simulink model "navigator"  (R2024b)
settings: Solver=FixedStepAuto  StartTime=0.0  StopTime=10.0  FixedStep=0.05  RelTol=1e-3
undefined symbols (not defined in the file or in its folder): CONSTANTS_RADIUS_OF_EARTH, GF_ACTION, GF_MAX_HOR_DIST, GF_MAX_VER_DIST
(part 2 of 2)

== stateflow chart navigator/Navigator ==
  state COMMAND [parallel]
    settings: executionOrder=1
    state CMD_DO_GO_AROUND [parallel]
      en:
      % 临时给输出赋值，后续删除
      o_pos_sp_triplet = i_pos_sp_triplet;
      o_mission_result.timestamp = uint64(getSimulationTime()*1e6);
      %
      settings: executionOrder=1
      state not_running
      state running
        en:
        publish_vehicle_command_ack(i_vehicle_command, VEHICLE_COMMAND.VEHICLE_CMD_RESULT_ACCEPTED);
      (default) -> COMMAND.CMD_DO_GO_AROUND.not_running
      COMMAND.CMD_DO_GO_AROUND.not_running -> COMMAND.CMD_DO_GO_AROUND.running : [i_vehicle_command.command == VEHICLE_COMMAND.VEHICLE_CMD_DO_GO_AROUND]
      COMMAND.CMD_DO_GO_AROUND.running -> COMMAND.CMD_DO_GO_AROUND.not_running : [i_vehicle_command.command ~= VEHICLE_COMMAND.VEHICLE_CMD_DO_GO_AROUND]
    state CMD_DO_REPOSITION [parallel]
      settings: executionOrder=2
      state not_running
      state running
        en:
        set_reposition_setpoint();
      (default) -> COMMAND.CMD_DO_REPOSITION.not_running
      COMMAND.CMD_DO_REPOSITION.not_running -> COMMAND.CMD_DO_REPOSITION.running : [i_vehicle_command.command == VEHICLE_COMMAND.VEHICLE_CMD_DO_REPOSITION ]
      COMMAND.CMD_DO_REPOSITION.running -> COMMAND.CMD_DO_REPOSITION.not_running : [i_vehicle_command.command ~= VEHICLE_COMMAND.VEHICLE_CMD_DO_REPOSITION]
    state CMD_NAV_TAKEOFF [parallel]
      settings: executionOrder=3
      state not_running
      state running
        en:
        % 前一航点
        if ((i_home_position.timestamp > 0) && i_home_position.valid_alt && i_home_position.valid_hpos && i_home_position.valid_lpos)
        g_takeoff_triplet.previous.valid = true;
        g_takeoff_triplet.previous.timestamp = uint64(getSimulationTime()*1e6);
        else
        g_takeoff_triplet.previous.valid = false;
        end
        g_takeoff_triplet.previous.lat = i_global_position.lat;
        g_takeoff_triplet.previous.lon = i_global_position.lon;
        g_takeoff_triplet.previous.alt = i_global_position.alt;
        g_takeoff_triplet.previous.yaw = i_local_position.heading;
        % 当前航点
        g_takeoff_triplet.current.valid = true;
        g_takeoff_triplet.current.timestamp = uint64(getSimulationTime()*1e6);
        g_takeoff_triplet.current.type = uint8(POSITION_SETPOINT.SETPOINT_TYPE_TAKEOFF);
        if isfinite(i_vehicle_command.param5) && isfinite(i_vehicle_command.param6)
        g_takeoff_triplet.current.lat = i_vehicle_command.param5;
        g_takeoff_triplet.current.lon = i_vehicle_command.param6;
        else
        g_takeoff_triplet.current.lat = i_global_position.lat;
        g_takeoff_triplet.current.lon = i_global_position.lon;
        end
        g_takeoff_triplet.current.alt = i_vehicle_command.param7;
        if ((i_home_position.timestamp > 0) && i_home_position.valid_alt && i_home_position.valid_hpos && i_home_position.valid_lpos)
        g_takeoff_triplet.current.yaw = i_vehicle_command.param4;
        else
        g_takeoff_triplet.current.yaw = i_local_position.heading;
        end
        g_takeoff_triplet.current.loiter_radius = NAV_LOITER_RAD;
        g_takeoff_triplet.current.loiter_direction = int8(1);
        % 下一航点
        g_takeoff_triplet.next.valid = false;
      (default) -> COMMAND.CMD_NAV_TAKEOFF.not_running
      COMMAND.CMD_NAV_TAKEOFF.not_running -> COMMAND.CMD_NAV_TAKEOFF.running : [i_vehicle_command.command == VEHICLE_COMMAND.VEHICLE_CMD_NAV_TAKEOFF]
      COMMAND.CMD_NAV_TAKEOFF.running -> COMMAND.CMD_NAV_TAKEOFF.not_running : [i_vehicle_command.command ~= VEHICLE_COMMAND.VEHICLE_CMD_NAV_TAKEOFF]
    state CMD_DO_CHANGE_SPEED [parallel]
      settings: executionOrder=4
      state not_running
      state running
        en:
        if (i_vehicle_command.param2 > eps)
        % 速度指令有效
        if (i_vehicle_status.vehicle_type == VEHICLE_STATUS.VEHICLE_TYPE_ROTARY_WING)
        g_mission_cruising_speed_mc = i_vehicle_command.param2;
        else
        g_mission_cruising_speed_fw = i_vehicle_command.param2;
        end
        else
        % 速度指令无效
        if (i_vehicle_status.vehicle_type == VEHICLE_STATUS.VEHICLE_TYPE_ROTARY_WING)
        g_mission_cruising_speed_mc = single(-1);
        else
        g_mission_cruising_speed_fw = single(-1);
        end
        % 设置油门指令
        if (i_vehicle_command.param3 > eps)
        g_mission_throttle = i_vehicle_command.param3 / 100;
        else
        g_mission_throttle = single(nan);
        end
        end
        publish_vehicle_command_ack(i_vehicle_command, VEHICLE_COMMAND.VEHICLE_CMD_RESULT_ACCEPTED);
      (default) -> COMMAND.CMD_DO_CHANGE_SPEED.not_running
      COMMAND.CMD_DO_CHANGE_SPEED.not_running -> COMMAND.CMD_DO_CHANGE_SPEED.running : [i_vehicle_command.command==VEHICLE_COMMAND.VEHICLE_CMD_DO_CHANGE_SPEED]
      COMMAND.CMD_DO_CHANGE_SPEED.running -> COMMAND.CMD_DO_CHANGE_SPEED.not_running : [i_vehicle_command.command~=VEHICLE_COMMAND.VEHICLE_CMD_DO_CHANGE_SPEED]
  state TRAFFIC [parallel]
    settings: executionOrder=2
  state GEOFENCE [parallel]
    settings: executionOrder=3
  state ACTION [parallel]
    en,du:
    switch uint8(i_vehicle_status.nav_state)
    case uint8(VEHICLE_STATUS.NAVIGATION_STATE_AUTO_MISSION)
    % g_pos_sp_triplet_published_invalid_once = false;
    % mission.set_execution_mode(mission_result_s::MISSION_EXECUTION_MODE_NORMAL);
    g_navigation_mode = VEHICLE_STATUS.NAVIGATION_STATE_AUTO_MISSION;
    case uint8(VEHICLE_STATUS.NAVIGATION_STATE_AUTO_LOITER)
    % g_pos_sp_triplet_published_invalid_once = false;
    g_navigation_mode = VEHICLE_STATUS.NAVIGATION_STATE_AUTO_LOITER;
    case uint8(VEHICLE_STATUS.NAVIGATION_STATE_AUTO_TAKEOFF)
    % g_pos_sp_triplet_published_invalid_once = false;
    g_navigation_mode = VEHICLE_STATUS.NAVIGATION_STATE_AUTO_TAKEOFF;
    case uint8(VEHICLE_STATUS.NAVIGATION_STATE_AUTO_LAND)
    % g_pos_sp_triplet_published_invalid_once = false;
    g_navigation_mode = VEHICLE_STATUS.NAVIGATION_STATE_AUTO_LAND;
    case uint8(VEHICLE_STATUS.NAVIGATION_STATE_AUTO_LANDENGFAIL)
    % g_pos_sp_triplet_published_invalid_once = false;
    g_navigation_mode = VEHICLE_STATUS.NAVIGATION_STATE_AUTO_LANDENGFAIL;
    case uint8(VEHICLE_STATUS.NAVIGATION_STATE_AUTO_LANDGPSFAIL)
    % g_pos_sp_triplet_published_invalid_once = false;
    g_navigation_mode = VEHICLE_STATUS.NAVIGATION_STATE_AUTO_LANDGPSFAIL;
    case uint8(VEHICLE_STATUS.NAVIGATION_STATE_AUTO_RTL)
    % g_pos_sp_triplet_published_invalid_once = false;
    % TODO
    otherwise
    g_navigation_mode = VEHICLE_STATUS.NAVIGATION_STATE_MAX;
    g_can_loiter_at_sp = false;
    end
    % 没有解锁不允许飞行
    if i_vehicle_status.arming_state ~= VEHICLE_STATUS.ARMING_STATE_ARMED
    g_navigation_mode = VEHICLE_STATUS.NAVIGATION_STATE_MAX;
    end
    % 记录当前导航状态
    %previous_nav_state = i_vehicle_status.nav_state;
    settings: executionOrder=4
    state LAND [parallel] [commented out]
      state on_disable [commented out]
      state on_active [commented out]
        state activation [commented out]
          en:
          set_land_item(true);
          o_mission_result.finished = false;
          g_mission_result_updated = true;
          % reset_mission_item_reached
          g_waypoint_position_reached = false;
          waypoint_yaw_reached_ = false;
          time_wp_reached_ = uint64(0);
          % convert mission item to current setpoint
          % 当前航点
          mission_item_ = NAV_STATE_ACTION.mission_apply_limitation(g_mission_item);
          NAV_STATE_ACTION.mission_item_to_position_setpoint(g_mission_item);
          % 前一航点
          o_pos_sp_triplet.previous.valid = false;
          % 下一航点
          o_pos_sp_triplet.next.valid = false;
          % 置标志位
          g_can_loiter_at_sp = false;
          g_pos_sp_triplet_updated = true;
        state active [commented out]
          en:
          % for VTOL update landing location during back transition
          o_pos_sp_triplet.current.lat = i_global_position.lat;
          o_pos_sp_triplet.current.lon = i_global_position.lon;
          g_pos_sp_triplet_updated = true;
        state Landed [commented out]
          en:
          o_mission_result.finished = true;
          g_mission_result_updated = true;
          NAV_STATE_ACTION.set_idle_item;
          NAV_STATE_ACTION.mission_item_to_position_setpoint(g_mission_item);
          g_pos_sp_triplet_updated = true;
        ACTION.LAND.on_active -> (junction 906) [commented out]
        (default) -> ACTION.LAND.on_active.activation [commented out]
        (junction 906) -> (junction 907) [commented out]
        (junction 906) -> ACTION.LAND.on_active.active [commented out] : % 飞机是vtol机型，并且处于过渡模式
            | [i_vehicle_status.is_vtol && i_vehicle_status.in_transition_mode]
        (junction 907) -> Landed [commented out] : % 飞机已经着陆
            | [land_detected.landed]
      (default) -> ACTION.LAND.on_disable [commented out]
      ACTION.LAND.on_disable -> ACTION.LAND.on_active [commented out] : [g_navigation_mode == NAVIGATION_MODE.land]
      ACTION.LAND.on_active -> ACTION.LAND.on_disable [commented out] : [g_navigation_mode ~= NAVIGATION_MODE.land]
    state LOITER [parallel] [commented out]
      state not_running [commented out]
        en,du:
        loiter_pos_set = false;
      state on_activation_active [commented out]
        state reposition [commented out]
          en:
          % rep的数据在navigator_main.cpp中处理
          o_pos_sp_triplet.current.velocity_valid = false;
          o_pos_sp_triplet.previous.yaw = i_local_position.heading;
          o_pos_sp_triplet.previous.lat = i_global_position.lat;
          o_pos_sp_triplet.previous.lon = i_global_position.lon;
          o_pos_sp_triplet.previous.alt = i_global_position.alt
          % 当前航路点用rep中表示
          o_pos_sp_triplet.current = g_reposition_triplet.current;
          % 下一个航路点无效
          o_pos_sp_triplet.next.valid = false;
          % 更新标志位
          g_can_loiter_at_sp = (o_pos_sp_triplet.current.type==POSITION_SETPOINT.SETPOINT_TYPE_LOITER);
          g_pos_sp_triplet_updated = true;
          % 设置reposition无效
          g_reposition_triplet.current.valid = false;
        state disarmed [commented out]
          en:
          loiter_pos_set = false;
        state set_loiter_pos [commented out]
          en:
          loiter_pos_set = true;
          % 若已着陆并上锁
          if ((i_vehicle_status.arming_state ~= VEHICLE_STATUS.ARMING_STATE_ARMED) && land_detected.landed)
          o_pos_sp_triplet.current.type = uint8(POSITION_SETPOINT.SETPOINT_TYPE_IDLE);
          g_can_loiter_at_sp = false;
          g_pos_sp_triplet_updated = true;
          loiter_pos_set = false;
          else
          g_mission_item.nav_cmd = uint16(NAVIGATION_CMD.NAV_CMD_LOITER_UNLIMITED);
          % set current mission item to loiter
          if (g_can_loiter_at_sp && o_pos_sp_triplet.current.valid)
          % 在当前的目标航点盘旋
          g_mission_item.lat = i_pos_sp_triplet.current.lat;
          g_mission_item.lon = i_pos_sp_triplet.current.lon;
          g_mission_item.altitude = i_pos_sp_triplet.current.alt;
          else
          % 在当前位置盘旋
          g_mission_item.lat = i_global_position.lat;
          g_mission_item.lon = i_global_position.lon;
          g_mission_item.altitude = i_global_position.alt;
          % （最小起飞高度 > 0 && item中的高度低于最小起飞的绝对高度），防止loiter高度在地面以下
          if (MIS_LTRMIN_ALT > 0) && (g_mission_item.altitude < i_home_position.alt + MIS_LTRMIN_ALT)
          g_mission_item.altitude = i_home_position.alt + MIS_LTRMIN_ALT;
          end
          end
          end
          g_mission_item.altitude_is_relative = false;
          g_mission_item.yaw = single(nan);
          g_mission_item.loiter_radius = NAV_LOITER_RAD;
          g_mission_item.acceptance_radius = navigator.get_acceptance_radius;
          g_mission_item.time_inside = single(0.0);
          g_mission_item.autocontinue = false;
          g_mission_item.origin = uint8(MISSION_ORIGIN.ONBOARD);
          % convert mission item to current setpoint
          o_pos_sp_triplet.previous.valid = false;
          % 当前航点
          o_pos_sp_triplet.current.velocity_valid = false;
          o_pos_sp_triplet.previous.velocity_valid = false;
          mission_item_ = NAV_STATE_ACTION.mission_apply_limitation(g_mission_item);
          NAV_STATE_ACTION.mission_item_to_position_setpoint(g_mission_item);
          %下一航点
          o_pos_sp_triplet.next.valid = false;
          % 更新标志位
          g_can_loiter_at_sp = (o_pos_sp_triplet.current.type==POSITION_SETPOINT.SETPOINT_TYPE_LOITER);
          g_pos_sp_triplet_updated = true;
        (default) -> (junction 846) [commented out]
        reposition -> reposition [commented out] : [g_reposition_triplet.current.valid]
        reposition -> disarmed [commented out] : [i_vehicle_status.arming_state ~= VEHICLE_STATUS.ARMING_STATE_ARMED]
        (junction 846) -> reposition [commented out] : [g_reposition_triplet.current.valid]
        (junction 846) -> (junction 847) [commented out]
        set_loiter_pos -> reposition [commented out] : [g_reposition_triplet.current.valid]
        (junction 847) -> set_loiter_pos [commented out]
      (default) -> ACTION.LOITER.not_running [commented out]
      ACTION.LOITER.not_running -> ACTION.LOITER.on_activation_active [commented out] : [g_navigation_mode == NAVIGATION_MODE.loiter]
      ACTION.LOITER.on_activation_active -> ACTION.LOITER.not_running [commented out] : [g_navigation_mode ~= NAVIGATION_MODE.loiter]
    state RTL [parallel] [commented out]
      state not_running [commented out]
        en,du:
        rtl_state = RTL_STATE.NONE;
        find_RTL_destination;
      state running [commented out]
        en:
        % TO DO: output RTL message, home / mission / safe point
        % 垂起旋翼阶段取消mission方式的降落，因为此处已经不是mission模式了
        deny_mission_landing_ = i_vehicle_status.is_vtol && (i_vehicle_status.vehicle_type == VEHICLE_STATUS.VEHICLE_TYPE_ROTARY_WING);
        get_rtl_alt_and_rad;
        print_des_type;
        state RTL_STATE_CLIMB [commented out]
          en:
          rtl_state = RTL_STATE.CLIMB;
          climb_and_return_done_ = false;
          g_can_loiter_at_sp = false;
          % 在当前位置爬升至指定高度
          if (i_vehicle_status.vehicle_type == VEHICLE_STATUS.VEHICLE_TYPE_ROTARY_WING)
          % 如果多旋翼则直接爬升到给定高度
          g_mission_item.nav_cmd = uint16(NAVIGATION_CMD.NAV_CMD_WAYPOINT);
          else
          %如果是固定翼，则盘旋上升到给定高度
          g_mission_item.nav_cmd = uint16(NAVIGATION_CMD.NAV_CMD_LOITER_TO_ALT);
          end
          g_mission_item.lat = i_global_position.lat;
          g_mission_item.lon = i_global_position.lon;
          g_mission_item.altitude = rtl_alt;
          g_mission_item.altitude_is_relative = false;
          g_mission_item.yaw = i_local_position.heading;
          g_mission_item.acceptance_radius = navigator.get_acceptance_radius;
          g_mission_item.time_inside = single(0);
          g_mission_item.autocontinue = true;
          g_mission_item.origin =uint8(MISSION_ORIGIN.ONBOARD);
          sprintf("RTL: climb to %f m (%f m above destination) \t", double(rtl_alt), double(rtl_alt - destination.alt))
          % mavlink_log_info(_navigator->get_mavlink_log_pub(), "RTL: climb to %d m (%d m above destination)\t",(int)ceilf(_rtl_alt), (int)ceilf(_rtl_alt - _destination.alt));
          % Reset all reached flags
          g_waypoint_position_reached = false;
          waypoint_yaw_reached_ = false;
          time_wp_reached_ = uint64(0);
          % TO DO: issue_command
          % 更新当前航点
          mission_item_ = NAV_STATE_ACTION.mission_apply_limitation(g_mission_item);
          NAV_STATE_ACTION.mission_item_to_position_setpoint(g_mission_item);
          g_pos_sp_triplet_updated = true;
        state RTL_STATE_RETURN [commented out]
          en:
          rtl_state = RTL_STATE.RETURN;
          climb_and_return_done_ = false;
          g_can_loiter_at_sp = false;
          % 返航至目标航点
          g_mission_item.nav_cmd = uint16(NAVIGATION_CMD.NAV_CMD_WAYPOINT);
          g_mission_item.lat = destination.lat;
          g_mission_item.lon = destination.lon;
          g_mission_item.altitude = rtl_alt;
          g_mission_item.altitude_is_relative = false;
          destination_dist = navigator.get_distance_2_next_waypoint(destination.lat, destination.lon, i_global_position.lat, i_global_position.lon);
          if (destination_dist < RTL_MIN_DIST)
          % 如果离着陆点很近，则采用着陆的航向
          g_mission_item.yaw = destination.yaw;
          else
          % 否则机头指向着陆点
          g_mission_item.yaw = navigator.get_bearing_2_next_waypoint(i_global_position.lat, i_global_position.lon, destination.lat, destination.lon);
          end
          g_mission_item.acceptance_radius = navigator.get_acceptance_radius;
          g_mission_item.time_inside = single(0);
          g_mission_item.autocontinue = true;
          g_mission_item.origin = uint8(MISSION_ORIGIN.ONBOARD);
          sprintf("RTL: return at %f m (%f m above destination) \t", double(g_mission_item.altitude), double(g_mission_item.altitude - destination.alt))
          % Reset all reached flags
          g_waypoint_position_reached = false;
          waypoint_yaw_reached_ = false;
          time_wp_reached_ = uint64(0);
          % TO DO: issue_command
          % 更新当前航点
          mission_item_ = NAV_STATE_ACTION.mission_apply_limitation(g_mission_item);
          NAV_STATE_ACTION.mission_item_to_position_setpoint(g_mission_item);
          g_pos_sp_triplet_updated = true;
        state RTL_STATE_DESCEND [commented out]
          en:
          rtl_state = RTL_STATE.DESCEND;
          climb_and_return_done_ = true;
          g_can_loiter_at_sp = false;
          % 下降至指定高度
          g_mission_item.nav_cmd = uint16(NAVIGATION_CMD.NAV_CMD_LOITER_TO_ALT);
          g_mission_item.lat = destination.lat;
          g_mission_item.lon = destination.lon;
          g_mission_item.altitude = min([destination.alt + RTL_DESCEND_ALT, i_global_position.alt, rtl_alt]);
          g_mission_item.altitude_is_relative = false;
          % Except for vtol which might be still off here and should point towards this location.
          d_current = navigator.get_distance_2_next_waypoint(i_global_position.lat, i_global_position.lon, g_mission_item.lat, g_mission_item.lon);
          if (i_vehicle_status.is_vtol && (d_current > navigator.get_acceptance_radius))
          g_mission_item.yaw = navigator.get_bearing_2_next_waypoint(i_global_position.lat, i_global_position.lon, g_mission_item.lat, g_mission_item.lon);
          else
          g_mission_item.yaw = destination.yaw;
          end
          if (i_vehicle_status.is_vtol)
          g_mission_item.loiter_radius = rtl_loiter_rad;
          end
          g_mission_item.acceptance_radius = navigator.get_acceptance_radius;
          g_mission_item.time_inside = single(0);
          g_mission_item.autocontinue = true;
          g_mission_item.origin = uint8(MISSION_ORIGIN.ONBOARD);
          % Disable previous setpoint to prevent drift.
          o_pos_sp_triplet.previous.valid = false;
          sprintf("RTL: descend to %f m (%f m above destination) \t", double(g_mission_item.altitude), double(g_mission_item.altitude - destination.alt))
          % Reset all reached flags
          g_waypoint_position_reached = false;
          waypoint_yaw_reached_ = false;
          time_wp_reached_ = uint64(0);
          % TO DO: issue_command
          % 更新当前航点
          mission_item_ = NAV_STATE_ACTION.mission_apply_limitation(g_mission_item);
          NAV_STATE_ACTION.mission_item_to_position_setpoint(g_mission_item);
          g_pos_sp_triplet_updated = true;
        state RTL_STATE_LOITER [commented out]
          en:
          rtl_state = RTL_STATE.LOITER;
          climb_and_return_done_ = true;
          g_can_loiter_at_sp = true;
          % Don't change altitude.
          g_mission_item.lat = destination.lat;
          g_mission_item.lon = destination.lon;
          g_mission_item.altitude = min([destination.alt + RTL_DESCEND_ALT, i_global_position.alt, rtl_alt]);
          g_mission_item.altitude_is_relative = false;
          g_mission_item.yaw = destination.yaw;
          g_mission_item.loiter_radius = NAV_LOITER_RAD;
          g_mission_item.acceptance_radius = navigator.get_acceptance_radius;
          g_mission_item.time_inside = max(RTL_LAND_DELAY, single(0.0));
          g_mission_item.autocontinue = (RTL_LAND_DELAY > eps);
          g_mission_item.origin = uint8(MISSION_ORIGIN.ONBOARD);
          if (RTL_LAND_DELAY > eps)
          g_mission_item.nav_cmd = uint16(NAVIGATION_CMD.NAV_CMD_LOITER_TIME_LIMIT)
          sprintf("RTL: loiter %f. \t", double(g_mission_item.time_inside));
          %mavlink_log_info(_navigator->get_mavlink_log_pub(), "RTL: loiter %.1fs\t", (double)get_time_inside(_mission_item));
          %events::send<float>(events::ID("rtl_loiter"), events::Log::Info, "RTL: loiter {1:.1}s", get_time_inside(_mission_item));
          else
          g_mission_item.nav_cmd = uint16(NAVIGATION_CMD.NAV_CMD_LOITER_UNLIMITED);
          sprintf("RTL: completed, loitering. \t")
          %mavlink_log_info(_navigator->get_mavlink_log_pub(), "RTL: completed, loitering\t");
          %events::send(events::ID("rtl_completed_loiter"), events::Log::Info, "RTL: completed, loitering");
          end
          % Reset all reached flags
          g_waypoint_position_reached = false;
          waypoint_yaw_reached_ = false;
          time_wp_reached_ = uint64(0);
          % TO DO: issue_command
          % 更新当前航点
          mission_item_ = NAV_STATE_ACTION.mission_apply_limitation(g_mission_item);
          NAV_STATE_ACTION.mission_item_to_position_setpoint(g_mission_item);
          g_pos_sp_triplet_updated = true;
        state RTL_STATE_LAND [commented out]
          en:
          rtl_state = RTL_STATE.LANDING;
          climb_and_return_done_ = true;
          g_can_loiter_at_sp = false;
          % Land at destination.
          g_mission_item.nav_cmd = uint16(NAVIGATION_CMD.NAV_CMD_LAND);
          g_mission_item.lat = destination.lat;
          g_mission_item.lon = destination.lon;
          g_mission_item.yaw = destination.yaw;
          g_mission_item.altitude = destination.alt;
          g_mission_item.altitude_is_relative = false;
          g_mission_item.acceptance_radius = navigator.get_acceptance_radius;
          g_mission_item.time_inside = single(0);
          g_mission_item.autocontinue = true;
          g_mission_item.origin = uint8(MISSION_ORIGIN.ONBOARD);
          %g_mission_item.land_precision = RTL_PLD_MD;
          %if (g_mission_item.land_precision == 1)
          %_navigator->get_precland()->set_mode(PrecLandMode::Opportunistic);
          %_navigator->get_precland()->on_activation();
          %elseif (g_mission_item.land_precision == 2)
          %_navigator->get_precland()->set_mode(PrecLandMode::Required);
          %_navigator->get_precland()->on_activation();
          %end
          sprintf("RTL: land at destination")
          %mavlink_log_info(_navigator->get_mavlink_log_pub(), "RTL: land at destination\t");
          % %events::send(events::ID("rtl_land_at_destination"), events::Log::Info, "RTL: land at destination");
          % Reset all reached flags
          g_waypoint_position_reached = false;
          waypoint_yaw_reached_ = false;
          time_wp_reached_ = uint64(0);
          % TO DO: issue_command
          % 更新当前航点
          mission_item_ = NAV_STATE_ACTION.mission_apply_limitation(g_mission_item);
          NAV_STATE_ACTION.mission_item_to_position_setpoint(g_mission_item);
          g_pos_sp_triplet_updated = true;
        state RTL_MOVE_TO_LAND_HOVER_VTOL [commented out]
          en:
          rtl_state = RTL_STATE.MOVE_TO_LAND_HOVER_VTOL;
          climb_and_return_done_ = true;
          g_can_loiter_at_sp = false;
          %
          g_mission_item.nav_cmd = uint16(NAVIGATION_CMD.NAV_CMD_WAYPOINT);
          g_mission_item.lat = destination.lat;
          g_mission_item.lon = destination.lon;
          g_mission_item.altitude = min([destination.alt + RTL_DESCEND_ALT, i_global_position.alt, rtl_alt]);
          g_mission_item.altitude_is_relative = false;
          g_mission_item.yaw = navigator.get_bearing_2_next_waypoint(i_global_position.lat, i_global_position.lon, g_mission_item.lat, g_mission_item.lon);
          g_mission_item.acceptance_radius = navigator.get_acceptance_radius;
          g_mission_item.origin = uint8(MISSION_ORIGIN.ONBOARD);
          % Reset all reached flags
          g_waypoint_position_reached = false;
          waypoint_yaw_reached_ = false;
          time_wp_reached_ = uint64(0);
          % TO DO: issue_command
          % 更新当前航点
          mission_item_ = NAV_STATE_ACTION.mission_apply_limitation(g_mission_item);
          NAV_STATE_ACTION.mission_item_to_position_setpoint(g_mission_item);
          g_pos_sp_triplet_updated = true;
        state RTL_STATE_TRANSITION_TO_MC [commented out]
          en:
          rtl_state = RTL_STATE.TRANSITION_TO_MC;
          climb_and_return_done_ = true;
          g_can_loiter_at_sp = false;
          % 设置固定翼切换到旋翼的过渡点
          g_mission_item.nav_cmd = uint16(NAVIGATION_CMD.NAV_CMD_DO_VTOL_TRANSITION);
          % params 是union联合体
          g_mission_item.time_inside = single(VTOL_VEHICLE_STATUS.VEHICLE_VTOL_STATE_MC);
          g_mission_item.acceptance_radius = single(0.0);
          g_mission_item.yaw = i_local_position.heading;
          g_mission_item.autocontinue = true;
          % Reset all reached flags
          g_waypoint_position_reached = false;
          waypoint_yaw_reached_ = false;
          time_wp_reached_ = uint64(0);
          % TO DO: issue_command
          % 更新当前航点
          mission_item_ = NAV_STATE_ACTION.mission_apply_limitation(g_mission_item);
          NAV_STATE_ACTION.mission_item_to_position_setpoint(g_mission_item);
          g_pos_sp_triplet_updated = true;
        state RTL_STATE_HEAD_TO_CENTER [commented out]
          en:
          rtl_state = RTL_STATE.HEAD_TO_CENTER;
          climb_and_return_done_ = true;
          g_can_loiter_at_sp = false;
          %
          g_mission_item.nav_cmd = uint16(NAVIGATION_CMD.NAV_CMD_WAYPOINT);
          g_mission_item.lat = destination.lat;
          g_mission_item.lon = destination.lon;
          g_mission_item.altitude = min([destination.alt + RTL_DESCEND_ALT, i_global_position.alt, rtl_alt]);
          g_mission_item.altitude_is_relative = false;
          g_mission_item.yaw = navigator.get_bearing_2_next_waypoint(i_global_position.lat, i_global_position.lon, g_mission_item.lat, g_mission_item.lon);
          g_mission_item.acceptance_radius = navigator.get_acceptance_radius;
          g_mission_item.time_inside = single(0);
          g_mission_item.autocontinue = true;
          g_mission_item.origin = uint8(MISSION_ORIGIN.ONBOARD);
          % Disable previous setpoint to prevent drift.
          o_pos_sp_triplet.previous.valid = false;
          % Reset all reached flags
          g_waypoint_position_reached = false;
          waypoint_yaw_reached_ = false;
          time_wp_reached_ = uint64(0);
          % TO DO: issue_command
          % 更新当前航点
          mission_item_ = NAV_STATE_ACTION.mission_apply_limitation(g_mission_item);
          NAV_STATE_ACTION.mission_item_to_position_setpoint(g_mission_item);
          g_pos_sp_triplet_updated = true;
        state RTL_STATE_LANDED [commented out]
          en:
          rtl_state = RTL_STATE.LANDED
          climb_and_return_done_ = true;
          g_can_loiter_at_sp = false;
          %
          NAV_STATE_ACTION.set_idle_item;
          rtl_alt_min_ = false;
          % Reset all reached flags
          g_waypoint_position_reached = false;
          waypoint_yaw_reached_ = false;
          time_wp_reached_ = uint64(0);
          % TO DO: issue_command
          % 更新当前航点
          mission_item_ = NAV_STATE_ACTION.mission_apply_limitation(g_mission_item);
          NAV_STATE_ACTION.mission_item_to_position_setpoint(g_mission_item);
          g_pos_sp_triplet_updated = true;
        (default) -> RTL_STATE_DESCEND [commented out] : % 如果rtl降落点类型为MISSION_LANDING，并且飞行器处于正在降落的过程中
            | [destination.type == RTL_DESTINATION_TYPE.MISSION_LANDING && ...
            | mission_landing_in_progress_]
        (default) -> RTL_STATE_CLIMB [commented out] : % 如果飞行器的高度低于预设的降落高度
            | [i_global_position.alt < ((destination.alt + RTL_RETURN_ALT) || ...
            | rtl_alt_min_)]
        (default) -> RTL_STATE_RETURN [commented out]
        RTL_STATE_CLIMB -> RTL_STATE_RETURN [commented out] : [NAV_STATE_ACTION.is_mission_item_reached(g_mission_item)]
        RTL_STATE_RETURN -> (junction 800) [commented out] : [NAV_STATE_ACTION.is_mission_item_reached(g_mission_item)]
        (junction 800) -> RTL_STATE_DESCEND [commented out] : [(RTL_LAND_DELAY < -0.01 || RTL_LAND_DELAY > 0.01) || ...
            | (i_vehicle_status.is_vtol && i_vehicle_status.vehicle_type == VEHICLE_STATUS.VEHICLE_TYPE_FIXED_WING)]
        (junction 800) -> (junction 801) [commented out]
        RTL_STATE_DESCEND -> (junction 802) [commented out] : [NAV_STATE_ACTION.is_mission_item_reached(g_mission_item)]
        (junction 802) -> (junction 801) [commented out]
        (junction 802) -> (junction 803) [commented out] : [i_vehicle_status.is_vtol && ...
            | i_vehicle_status.vehicle_type == VEHICLE_STATUS.VEHICLE_TYPE_FIXED_WING]
        (junction 801) -> (junction 805) [commented out]
        (junction 802) -> RTL_STATE_LOITER [commented out] : [RTL_LAND_DELAY < -0.01 || RTL_LAND_DELAY > 0.01]
        (junction 803) -> RTL_STATE_HEAD_TO_CENTER [commented out]
        RTL_STATE_LOITER -> (junction 805) [commented out] : [NAV_STATE_ACTION.is_mission_item_reached(g_mission_item)]
        (junction 805) -> (junction 804) [commented out]
        (junction 804) -> RTL_STATE_LAND [commented out]
        RTL_STATE_TRANSITION_TO_MC -> RTL_MOVE_TO_LAND_HOVER_VTOL [commented out] : [NAV_STATE_ACTION.is_mission_item_reached(g_mission_item)]
        RTL_MOVE_TO_LAND_HOVER_VTOL -> RTL_STATE_LAND [commented out] : [NAV_STATE_ACTION.is_mission_item_reached(g_mission_item)]
        RTL_STATE_HEAD_TO_CENTER -> RTL_STATE_TRANSITION_TO_MC [commented out] : [NAV_STATE_ACTION.is_mission_item_reached(g_mission_item)]
        RTL_STATE_LAND -> RTL_STATE_LANDED [commented out] : [NAV_STATE_ACTION.is_mission_item_reached(g_mission_item)]
        (default) -> RTL_STATE_LANDED [commented out] : % 飞行器已经着陆
            | [land_detected.landed]
      (default) -> ACTION.RTL.not_running [commented out]
      ACTION.RTL.not_running -> ACTION.RTL.running [commented out] : [g_navigation_mode == NAVIGATION_MODE.rtl]
      ACTION.RTL.running -> ACTION.RTL.not_running [commented out] : [g_navigation_mode ~= NAVIGATION_MODE.rtl]
    state TAKEOFF [parallel]
      settings: executionOrder=1
      state on_disable
      state on_active
        state takeoff_entry
          en:
          set_takeoff_position()
        state takeoff_finished
          en:
          set_takeoff_finished()
        (default) -> takeoff_entry
        takeoff_finished -> takeoff_entry : [g_takeoff_triplet.current.valid]
        takeoff_entry -> takeoff_finished : [is_mission_item_reached()]
      (default) -> ACTION.TAKEOFF.on_disable
      ACTION.TAKEOFF.on_disable -> ACTION.TAKEOFF.on_active : [g_navigation_mode==VEHICLE_STATUS.NAVIGATION_STATE_AUTO_TAKEOFF]
      ACTION.TAKEOFF.on_active -> ACTION.TAKEOFF.on_disable : [g_navigation_mode~=VEHICLE_STATUS.NAVIGATION_STATE_AUTO_TAKEOFF]
    state ENGINE_FAILURE [parallel] [commented out]
      state not_running [commented out]
        en,du:
        % ef_state: engine failure state
        ef_state = EFSTATE.EF_STATE_NONE;
      state on_activation_active [commented out]
        state activation [commented out]
          en:
          ef_state = EFSTATE.EF_STATE_NONE;
          advance_ef;
          set_ef_item;
        state active [commented out]
          en:
          advance_ef;
          set_ef_item;
        ACTION.ENGINE_FAILURE.on_activation_active -> ACTION.ENGINE_FAILURE.on_activation_active.active [commented out] : [NAV_STATE_ACTION.is_mission_item_reached(g_mission_item)]
        (default) -> ACTION.ENGINE_FAILURE.on_activation_active.activation [commented out]
      (default) -> ACTION.ENGINE_FAILURE.not_running [commented out]
      ACTION.ENGINE_FAILURE.not_running -> ACTION.ENGINE_FAILURE.on_activation_active [commented out] : [g_navigation_mode == NAVIGATION_MODE.engineFailure]
      ACTION.ENGINE_FAILURE.on_activation_active -> ACTION.ENGINE_FAILURE.not_running [commented out] : [g_navigation_mode ~= NAVIGATION_MODE.engineFailure]
    state MISSION [parallel] [commented out]
      state not_running [commented out]
      state running [commented out]
        en:
      (default) -> ACTION.MISSION.not_running [commented out]
      ACTION.MISSION.not_running -> ACTION.MISSION.running [commented out] : [g_navigation_mode == NAVIGATION_MODE.mission]
      ACTION.MISSION.running -> ACTION.MISSION.not_running [commented out] : [g_navigation_mode ~= NAVIGATION_MODE.mission]
    state GPS_FAILURE [parallel] [commented out]
      state not_running [commented out]
        en,du:
        % 仅在setpoint移动时重置GPS_FAILURE状态
        if (~g_can_loiter_at_sp)
        gpsf_state = GPSFSTATE.GPSF_STATE_NONE;
        end
      state on_activation_active [commented out]
        state activation [commented out]
          en:
          gpsf_state = GPSFSTATE.GPSF_STATE_NONE;
          timestamp_activation = uint64(getSimulationTime()*1e6);
          advance_gpsf;
          set_gpsf_item;
        state active [commented out]
          en:
          switch (gpsf_state)
          case GPSFSTATE.GPSF_STATE_LOITER
          % 在这种情况下，不会运行位置控制器；所以navigator在这里发布姿态的setpoint
          % att_sp.timestamp = uint64(getSimulationTime()*1e6);
          % att_sp.roll_body = single(deg2rad(NAV_GPSF_R));
          % att_sp.pitch_body = single(deg2rad(NAV_GPSF_P));
          % att_sp.thrust_body(1) = NAV_GPSF_TR;
          % att_sp.q_d = euler_to_quat(att_sp.roll_body, att_sp.pitch_body, 0);
          % TO DO: publish att_sp
          %
          % measure time
          if (NAV_GPSF_LT > eps) && ((uint64(getSimulationTime()*1e6) - timestamp_activation) > NAV_GPSF_LT)
          sprintf("GPS not recovered, switching to next failure state. \n")
          advance_gpsf;
          end
          case GPSFSTATE.GPSF_STATE_TERMINATE
          set_gpsf_item;
          advance_gpsf;
          otherwise
          end
        ACTION.GPS_FAILURE.on_activation_active -> ACTION.GPS_FAILURE.on_activation_active.active [commented out]
        (default) -> ACTION.GPS_FAILURE.on_activation_active.activation [commented out]
      (default) -> ACTION.GPS_FAILURE.not_running [commented out]
      ACTION.GPS_FAILURE.not_running -> ACTION.GPS_FAILURE.on_activation_active [commented out] : [g_navigation_mode == NAVIGATION_MODE.gpsFailure]
      ACTION.GPS_FAILURE.on_activation_active -> ACTION.GPS_FAILURE.not_running [commented out] : [g_navigation_mode ~= NAVIGATION_MODE.gpsFailure]
  data: phi function_input; theta function_input; psi function_input; q0 function_output; q1 function_output; q2 function_output; q3 function_output; lat function_input; lon function_input; alt function_input; inside function_output; at_current_location function_input; loiter_pos_set local boolean size=1 =false; destination_check_time local uint64 size=1 =uint64(0); destination_dist local single; d_current local single size=1; rtl_state local Enum: PX4_RTL_STATE size=1; rtl_loiter_rad local single size=1; rtl_alt local single size=1; destination local Bus: px4_rtl_position size=1; deny_mission_landing_ local boolean size=1 =false; mission_landing_in_progress_ local boolean size=1 =false; climb_and_return_done_ local boolean size=1 =false; ef_state local Enum: PX4_EFSTATE size=1; destination_check_time local uint64 size=1 =uint64(0); rtl_state local Enum: PX4_RTL_STATE size=1; rtl_loiter_rad local single size=1; rtl_alt local single size=1; destination local Bus: px4_rtl_position; gpsf_state local Enum: PX4_GPSFSTATE size=1; timestamp_activation local uint64 size=1; time function_output; item function_input; abs_altitude function_input; alt function_output; isreached function_output; min_clearance function_input; item function_output; at_current_location function_input; g_waypoint_position_reached local boolean size=1 =false; waypoint_yaw_reached_ local boolean size=1 =false; time_wp_reached_ local uint64 size=1 =uint64(0); lat_now function_input; lon_now function_input; lat_next function_input; lon_next function_input; dist function_output; lat_now function_input; lon_now function_input; lat_next function_input; lon_next function_input; bearing function_output; speed function_output; radius function_output; radius function_output single; speed function_input; radius function_output single; radius function_output; radius function_output; mission_item_yaw function_input; yaw function_output; cmd function_input; result function_input; throttle function_output single; i_vehicle_command input Bus: vehicle_command_s size=1; i_global_position input Bus: vehicle_global_position_s size=1; i_local_position input Bus: vehicle_local_position_s size=1; i_vehicle_status input Bus: vehicle_status_s size=1; RTL_RETURN_ALT parameter size=1; RTL_CONE_ANG parameter size=1; RTL_LOITER_RAD parameter size=1; NAV_ACC_RAD parameter size=1; g_pos_sp_triplet_updated local boolean size=1; i_land_detected input Bus: vehicle_land_detected_s size=1; i_pos_sp_triplet input Bus: position_setpoint_triplet_s size=1; i_home_position input Bus: home_position_s size=1; NAV_LOITER_RAD parameter size=1; i_pos_ctrl_status input Bus: position_controller_status_s size=1; o_pos_sp_triplet output Bus: position_setpoint_triplet_s size=1; MIS_LTRMIN_ALT parameter size=1; g_mission_throttle local single size=1 =single(nan); g_mission_cruising_speed_mc local single size=1 =single(-1.0); g_mission_cruising_speed_fw local single size=1 =single(-1.0); g_reposition_triplet local Bus: position_setpoint_triplet_s size=1; g_takeoff_triplet local Bus: position_setpoint_triplet_s size=1; MIS_TAKEOFF_ALT parameter size=1; o_mission_result output Bus: mission_result_s size=1; NAV_GPSF_R parameter size=1; NAV_GPSF_P parameter size=1; NAV_GPSF_TR parameter size=1; NAV_GPSF_LT parameter size=1; CONSTANTS_RADIUS_OF_EARTH parameter single size=1; RTL_MIN_DIST parameter single size=1; g_rtl_alt_min local boolean size=1 =false; RTL_DESCEND_ALT parameter size=1; RTL_LAND_DELAY parameter size=1; RTL_PLD_MD parameter size=1; RTL_TYPE parameter size=1; VT_B_DEC_MSS parameter size=1; VT_B_REV_DEL parameter size=1; MIS_YAW_ERR parameter size=1; MIS_YAW_TMT parameter size=1; NAV_FW_ALTL_RAD parameter size=1; NAV_FW_ALT_RAD parameter size=1; NAV_MC_ALT_RAD parameter size=1; GF_ACTION parameter size=1; MPC_JERK_AUTO parameter size=1; MPC_ACC_HOR parameter size=1; g_navigation_mode local Enum: VEHICLE_STATUS size=1; g_mission_item local Bus: mission_route_point_s size=1; g_mission_result_updated local boolean size=1 =false; g_can_loiter_at_sp local boolean size=1 =false; o_command_ack output Bus: vehicle_command_ack_s; MISSION_ORIGIN_ONBOARD constant uint8 size=1 =1; MISSION_ORIGIN_MAVLINK constant uint8 size=1 =0
  function [q0,q1,q2,q3] = eul_to_quat(phi,theta,psi):
    | function [q0,q1,q2,q3] = eul_to_quat(phi,theta,psi)
    | [q0,q1,q2,q3] = euler2quat(phi,theta,psi);
    | end
  function set_reposition_setpoint:
    | function set_reposition_setpoint
    | 
    | %% 判断reposition是否在禁飞区内
    | reposition_valid = true;
    | if (GF_ACTION ~= GEOFENCE_RESULT.GF_ACTION_NONE &&  GF_ACTION ~= GEOFENCE_RESULT.GF_ACTION_WARN)
    |     if isfinite(i_vehicle_command.param5) && isfinite(i_vehicle_command.param6)
    |         lat = i_vehicle_command.param5;
    |         lon = i_vehicle_command.param6;
    | 
    |         if isfinite(i_vehicle_command.param7)
    |             alt = i_vehicle_command.param7;
    |         else
    |             alt = i_global_position.alt;
    |         end
    | 
    |         reposition_valid = GEOFENCE.checkAll(lat, lon, alt);
    |     end
    | end
    | 
    | if ~reposition_valid
    |     %mavlink_log_critical(&_mavlink_log_pub, "Reposition is outside geofence\t");
    |     %events::send(events::ID("navigator_reposition_outside_geofence"), {events::Log::Error, events::LogInternal::Info},
    |     %"Reposition is outside geofence");
    | end
    | 
    | %% 初始化上个航点
    | g_reposition_triplet.previous.valid = true;
    | g_reposition_triplet.previous.timestamp = uint64(getSimulationTime()*1e6);
    | g_reposition_triplet.previous.lat = i_global_position.lat;
    | g_reposition_triplet.previous.lon = i_global_position.lon;
    | g_reposition_triplet.previous.alt = i_global_position.alt;
    | g_reposition_triplet.previous.yaw = i_local_position.heading;
    | 
    | %% 初始化当前航点
    | g_reposition_triplet.current.valid = true;
    | g_reposition_triplet.current.timestamp = uint64(getSimulationTime()*1e6);
    | g_reposition_triplet.current.loiter_radius = NAV_LOITER_RAD;
    | g_reposition_triplet.current.loiter_direction = int8(1);
    | g_reposition_triplet.current.type = uint8(POSITION_SETPOINT.SETPOINT_TYPE_LOITER);
    | 
    | % 如果没有速度参数，使用默认值
    | if (i_vehicle_command.param1 <= 0 || ~isfinite(i_vehicle_command.param1))
    |     g_reposition_triplet.current.cruising_speed = get_cruising_speed();
    | else
    |     g_reposition_triplet.current.cruising_speed = i_vehicle_command.param1;
    | end
    | % 油门
    | g_reposition_triplet.current.cruising_throttle = get_cruising_throttle();
    | % 提前量
    | g_reposition_triplet.current.acceptance_radius = get_acceptance_radius();
    | % 偏航角
    | if isfinite(i_vehicle_command.param4)
    |     g_reposition_triplet.current.yaw = i_vehicle_command.param4;
    |     g_reposition_triplet.current.yaw_valid = true;
    | else
    |     g_reposition_triplet.current.yaw = single(nan);
    |     g_reposition_triplet.current.yaw_valid = false;
    | end
    | % 经纬高
    | if isfinite(i_vehicle_command.param5) && isfinite(i_vehicle_command.param6)
    |     % 经纬度有效
    |     g_reposition_triplet.current.lat = i_vehicle_command.param5;
    |     g_reposition_triplet.current.lon = i_vehicle_command.param6;
    |     if isfinite(i_vehicle_command.param7)
    |         g_reposition_triplet.current.alt = i_vehicle_command.param7;
    |     else
    |         g_reposition_triplet.current.alt = i_global_position.alt;
    |     end
    | elseif i_vehicle_command.param7
    |     % 经纬度无效，高度有效
    |     g_reposition_triplet.current.lat = i_pos_sp_triplet.current.lat;
    |     g_reposition_triplet.current.lon = i_pos_sp_triplet.current.lon;
    |     g_reposition_triplet.current.alt = i_vehicle_command.param7;
    | else
    |     % 经纬高均无效
    |     g_reposition_triplet.current.alt = i_global_position.alt;
    | 
    |     if i_vehicle_status.vehicle_type == VEHICLE_STATUS.VEHICLE_TYPE_ROTARY_WING && i_pos_sp_triplet.current.type ~= uint8(POSITION_SETPOINT.SETPOINT_TYPE_TAKEOFF)
    |         % 多旋翼计算刹车距离，确定悬停位置
    |         course_over_ground = atan2(i_local_position.vy, i_local_position.vx);
    |         velocity_hor_abs = sqrt(i_local_position.vx^2 + i_local_position.vy^2);
    |         multirotor_braking_distance = velocity_hor_abs * (velocity_hor_abs / (2 * MPC_ACC_HOR) + (0.6 * MPC_JERK_AUTO) / MPC_JERK_AUTO);
    | 
    |         [g_reposition_triplet.current.lat, g_reposition_triplet.current.lon] = waypoint_from_heading_and_distance(i_global_position.lat, i_global_position.lon,...
    |             course_over_ground, multirotor_braking_distance);
    |         g_reposition_triplet.current.yaw = i_local_position.heading;
    |         g_reposition_triplet.current.yaw_valid = true;
    |     else
    |         % 固定翼使用当前位置进行盘旋
    |         g_reposition_triplet.current.lat = i_global_position.lat;
    |         g_reposition_triplet.current.lon = i_global_position.lon;
    |     end
    | end
    | 
    | %% 初始化下个航点
    | g_reposition_triplet.next.valid = false;
    | 
    | end
  function inside = checkAll(lat, lon, alt):
    | function inside = checkAll(lat, lon, alt)
    | 
    | inside = false;
  function set_land_item(at_current_location):
    | % set current mission item to Land
    | function set_land_item(at_current_location)
    | 
    | % VTOL transition to RW before landing
    | % 对于vtol机型，降落前需要转换为旋翼
    | % if navigator->force_vtol()
    | %     vcmd.command = NAV_CMD_DO_VTOL_TRANSITION;
    | %     vcmd.param1 = vtol_vehicle_status_s::VEHICLE_VTOL_STATE_MC;
    | %     vcmd.param2 = 0.0f;
    | %     _navigator->publish_vehicle_cmd(&vcmd);
    | % end
    | 
    | % set the land item
    | g_mission_item.nav_cmd = uint16(NAVIGATION_CMD.NAV_CMD_LAND);
    | 
    | if at_current_location
    |     % use current position
    |     g_mission_item.lat = double(nan); % descend at current position
    |     g_mission_item.lon = double(nan);
    |     g_mission_item.yaw = i_local_position.heading;
    | else
    |     % use home position
    |     g_mission_item.lat = i_home_position.lat;
    |     g_mission_item.lon = i_home_position.lon;
    |     g_mission_item.yaw = i_home_position.yaw;
    | end
    | 
    | g_mission_item.altitude = single(0.0);
    | g_mission_item.altitude_is_relative = false;
    | g_mission_item.loiter_radius = NAV_LOITER_RAD;
    | g_mission_item.acceptance_radius = navigator.get_acceptance_radius;
    | g_mission_item.time_inside = single(0.0);
    | g_mission_item.autocontinue = true;
    | g_mission_item.origin = uint8(MISSION_ORIGIN.ONBOARD);
    | 
    | end
  function find_RTL_destination:
    | function find_RTL_destination
    | 
    | destination = initial;
    | 
    | 
    | % if (getSimulationTime - destination_check_time) >= 1 && (i_home_position.timestamp > 0) && i_home_position.valid_alt && i_home_position.valid_hpos && i_home_position.valid_lpos
    | %     destination_check_time = getSimulationTime;
    | %     
    | %     % set destination to home per default, then check if other valid landing spot is closer
    | %     destination.lat = i_home_position.lat;
    | %     destination.lon = i_home_position.lon;
    | %     destination.alt = i_home_position.alt;
    | %     destination.yaw = i_home_position.yaw;
    | %     destination.safe_point_index = uint8(0);
    | %     destination.type = uint8(RTL_DESTINATION_TYPE.HOME);
    | %     
    | %     lon_scale = cos(deg2rad(i_global_position.lat));
    | %     
    | %     % get distance to home position
    | %     dlat = i_home_position.lat - i_global_position.lat;
    | %     dlon = i_home_position.lon - i_global_position.lon;
    | %     min_dist_squared = coord_dist_sq(dlat, dlon, lon_scale);
    | %     
    | %     % consider the mission landing if not RTL_HOME type set
    | %     if (RTL_TYPE ~= RTL_TYPE.HOME) && land_start_available_
    | %         if i_vehicle_status.is_vtol && (i_vehicle_status.vehicle_type == VEHICLE_STATUS.VEHICLE_TYPE_ROTARY_WING)
    | %             mission_landing_lat = landing_lat_;
    | %             mission_landing_lon = landing_lon_;
    | %             mission_landing_alt = landing_alt_;
    | %             destination_type = uint8(RTL_DESTINATION_TYPE.HOME);
    | %         else
    | %             mission_landing_lat = landing_start_lat_;
    | %             mission_landing_lon = landing_start_lon_;
    | %             mission_landing_alt = landing_start_alt_;
    | %             destination_type = uint8(RTL_DESTINATION_TYPE.MISSION_LANDING);
    | %         end
    | %         
    | %         % compare home position to landing position to decide which is closer
    | %         dlat = mission_landing_lat - i_global_position.lat;
    | %         dlon = mission_landing_lon - i_global_position.lon;
    | %         dist_squared = coord_dist_sq(dlat, dlon, lon_scale);
    | %         
    | %         if (dist_squared < min_dist_squared) || (RTL_TYPE ~= RTL_TYPE.CLOSEST)
    | %             min_dist_squared = dist_squared;
    | %             destination.lat = mission_landing_lat;
    | %             destination.lon = mission_landing_lon;
    | %             destination.alt = mission_landing_alt;
    | %             destination.type = destination_type;
    | %         end
    | %     end
    | %     
    | %     % 涉及到航点读取，未做
    | % end
    | 
    | end
    | 
    | 
    | %% 
    | function out = initial
    | out.lat = i_home_position.lat;
    | out.lon = i_home_position.lon;
    | out.alt = i_home_position.alt;
    | out.yaw = i_home_position.yaw;
    | out.safe_point_index = uint8(0);
    | out.type = uint8(RTL_DESTINATION_TYPE.HOME);
    | end
    | 
    | 
    | %% 
    | function out = coord_dist_sq(lat_diff,lon_diff,lon_scale)
    | 
    | lon_diff_scaled = lon_scale * wrap(lon_diff, -180, 180);
    | out = lat_diff * lat_diff + lon_diff_scaled * lon_diff_scaled;
    | 
    | end
  function get_rtl_alt_and_rad:
    |      function get_rtl_alt_and_rad
    | 
    | % 默认盘旋半径
    | % RTL_LOITER_RAD = 1;
    | % RTL_CONE_ANG = 1;
    | rtl_loiter_rad = RTL_LOITER_RAD;
    | 
    | % 根据处于旋翼阶段还是固定翼阶段，返回rtl高度
    | if i_vehicle_status.vehicle_type == VEHICLE_STATUS.VEHICLE_TYPE_ROTARY_WING
    |     rtl_alt = calculate_return_alt_from_cone_half_angle(RTL_CONE_ANG);
    | else
    |     rtl_alt = max([i_global_position.alt, destination.alt, i_home_position.alt + RTL_RETURN_ALT]);
    | end
    | 
    | end
    | 
    | %% 旋翼飞机或旋翼阶段飞机的rtl高度
    | function alt = calculate_return_alt_from_cone_half_angle(cone_half_angle_deg)
    | 
    | % horizontal distance to destination
    | % 计算飞机到降落点的水平距离
    | destination_dist = get_distance_to_next_waypoint(destination.lat, destination.lon, i_global_position.lat, i_global_position.lon);
    | 
    | % minium rtl altitude to use when outside of horizontal acceptance radius of target position.
    | % We choose the minimum height to be two times the distance from the land position in order to
    | % avoid the vehicle touching the ground while still moving horizontally.
    | % 在目标位置的水平接受半径外使用的rtl高度。我们选择最小高度的距离是距离土地位置的两倍,以避免车辆在地面移动时触碰地面。
    | return_altitude_min_outside_acceptance_rad_amsl = destination.alt + 2.0 * get_acceptance_radius;
    | 
    | return_altitude_amsl = destination.alt + RTL_RETURN_ALT;
    | 
    | if (destination_dist <= get_acceptance_radius)
    |     return_altitude_amsl = destination.alt + 2.0 * destination_dist;   
    | else
    |     if (cone_half_angle_deg > 0) && (destination_dist <= RTL_MIN_DIST)
    |         
    |         % constrain cone half angle to meaningful values. All other cases are already handled above.
    |         cone_half_angle_rad = deg2rad(constrain(cone_half_angle_deg, 1, 89));
    |         
    |         % minimum altitude we need in order to be within the user defined cone
    |         cone_intersection_altitude_amsl = destination_dist / tan(cone_half_angle_rad) + destination.alt;
    |         
    |         return_altitude_amsl = min(cone_intersection_altitude_amsl, return_altitude_amsl);
    |     end
    |     
    |     return_altitude_amsl = max(return_altitude_amsl, return_altitude_min_outside_acceptance_rad_amsl);
    | end
    | 
    | alt = max(return_altitude_amsl, i_global_position.alt);
    | 
    | end
  function print_des_type:
    | function print_des_type
    | 
    | % 打印rtl目的点的类型
    | % output the correct message, depending on where the RTL destination is
    | switch (uint8(destination.type))
    |     case uint8(RTL_DESTINATION_TYPE.HOME)
    |         sprintf("RTL: landing at home position.");
    |         
    |     case uint8(RTL_DESTINATION_TYPE.MISSION_LANDING)
    |         sprintf("RTL: landing at mission landing.");
    |         
    |     case uint8(RTL_DESTINATION_TYPE.SAFE_POINT)
    |         sprintf("RTL: landing at safe landing point.");
    | end
    |         
    | end
  function set_takeoff_position:
    | function set_takeoff_position()
    | 
    | %% 确定默认的起飞高度
    | % 如果home点有效，起飞高度为home点的海平面高度加上起飞的最小高度
    | if ((i_home_position.timestamp > 0) && i_home_position.valid_alt && i_home_position.valid_hpos && i_home_position.valid_lpos)
    |     min_abs_altitude = i_global_position.alt + MIS_TAKEOFF_ALT;
    | else
    |     min_abs_altitude = MIS_TAKEOFF_ALT;
    | end
    | 
    | %% 如果用户设置了起飞高度
    | % g_takeoff_triplet是在navigator_main.cpp中通过获取cmd参数得到的lat,lon,alt
    | if (g_takeoff_triplet.current.valid && isfinite(g_takeoff_triplet.current.alt) && ...
    |         (i_home_position.timestamp > 0) && i_home_position.valid_alt && i_home_position.valid_hpos && i_home_position.valid_lpos)
    |     % 使用用户设置的起飞高度
    |     abs_altitude = g_takeoff_triplet.current.alt;
    |     if (abs_altitude < min_abs_altitude)
    |         abs_altitude = min_abs_altitude;
    |     end
    |     sprintf("Using minimum takeoff altitude: %f m", double(MIS_TAKEOFF_ALT))
    |     % mavlink_log_critical
    | else
    |     abs_altitude = min_abs_altitude;
    |     sprintf("Using minimum takeoff altitude: %f m", double(MIS_TAKEOFF_ALT))
    |     % mavlink_log_info
    | end
    | 
    | if (abs_altitude < i_global_position.alt)
    |     % If the suggestion is lower than our current alt, let's not go down
    |     abs_altitude = i_global_position.alt;
    |     sprintf("Already higher than takeoff altitude")
    | end
    | 
    | set_takeoff_item(abs_altitude);
    | 
    | o_mission_result.finished = false;
    | g_mission_result_updated = true;
    | g_waypoint_position_reached = false;
    | waypoint_yaw_reached_ = false;
    | time_wp_reached_ = uint64(0);
    | 
    | % convert mission item to current setpoint
    | mission_apply_limitation();
    | mission_item_to_position_setpoint();
    | o_pos_sp_triplet.current.yaw_valid = true;
    | 
    | if g_takeoff_triplet.current.valid
    |     o_pos_sp_triplet.current.lat = g_takeoff_triplet.current.lat;
    |     o_pos_sp_triplet.current.lon = g_takeoff_triplet.current.lon;
    |     if isfinite(g_takeoff_triplet.current.yaw)
    |         o_pos_sp_triplet.current.yaw =  o_pos_sp_triplet.current.yaw;
    |     end
    |     g_takeoff_triplet.current.valid = false;
    | end
    | 
    | % 前一航点
    | o_pos_sp_triplet.previous.valid = false;
    | % 下一航点
    | o_pos_sp_triplet.next.valid = false;
    | 
    | % 置标志位
    | if (isfinite(o_pos_sp_triplet.current.lat) && isfinite(o_pos_sp_triplet.current.lon))
    |     g_can_loiter_at_sp = true;
    | else
    |     g_can_loiter_at_sp = false;
    | end
    | 
    | g_pos_sp_triplet_updated = true;
    | 
    | end
    | 
    | %% 设置takeoff_item
    | function set_takeoff_item(alt)
    | 
    | g_mission_item.nav_cmd = uint16(NAVIGATION_CMD.NAV_CMD_TAKEOFF);
    | g_mission_item.lat = i_global_position.lat;
    | g_mission_item.lon = i_global_position.lon;
    | g_mission_item.yaw = i_local_position.heading;
    | g_mission_item.altitude = alt;
    | g_mission_item.altitude_is_relative = false;
    | g_mission_item.loiter_radius = NAV_LOITER_RAD;
    | g_mission_item.autocontinue = false;
    | g_mission_item.origin = uint8(MISSION_ORIGIN.ONBOARD);
    | 
    | end
  function set_takeoff_finished:
    | function set_takeoff_finished
    | 
    | %% 确定默认的起飞高度
    | % 如果home点有效，起飞高度为home点的海平面高度加上起飞的最小高度
    | if ((i_home_position.timestamp > 0) && i_home_position.valid_alt && i_home_position.valid_hpos && i_home_position.valid_lpos)
    |     min_abs_altitude = i_global_position.alt + MIS_TAKEOFF_ALT;
    | else
    |     min_abs_altitude = MIS_TAKEOFF_ALT;
    | end
    | 
    | %% 如果用户设置了起飞高度
    | % g_takeoff_triplet是在navigator_main.cpp中通过获取cmd参数得到的lat,lon,alt
    | if (g_takeoff_triplet.current.valid && isfinite(g_takeoff_triplet.current.alt) && ...
    |         (i_home_position.timestamp > 0) && i_home_position.valid_alt && i_home_position.valid_hpos && i_home_position.valid_lpos)
    |     % 使用用户设置的起飞高度
    |     abs_altitude = g_takeoff_triplet.current.alt;
    |     if (abs_altitude < min_abs_altitude)
    |         abs_altitude = min_abs_altitude;
    |     end
    |     sprintf("Using minimum takeoff altitude: %f m", double(MIS_TAKEOFF_ALT))
    |     % mavlink_log_critical
    | else
    |     abs_altitude = min_abs_altitude;
    |     sprintf("Using minimum takeoff altitude: %f m", double(MIS_TAKEOFF_ALT))
    |     % mavlink_log_info
    | end
    | 
    | if (abs_altitude < i_global_position.alt)
    |     % If the suggestion is lower than our current alt, let's not go down
    |     abs_altitude = i_global_position.alt;
    |     sprintf("Already higher than takeoff altitude")
    | end
    | 
    | set_takeoff_item(abs_altitude);
    | 
    | o_mission_result.finished = false;
    | g_mission_result_updated = true;
    | g_waypoint_position_reached = false;
    | waypoint_yaw_reached_ = false;
    | time_wp_reached_ = uint64(0);
    | 
    | % convert mission item to current setpoint
    | mission_item_ = mission_apply_limitation(g_mission_item);
    | mission_item_to_position_setpoint(g_mission_item);
    | o_pos_sp_triplet.current.yaw_valid = true;
    | 
    | if g_takeoff_triplet.current.valid
    |     o_pos_sp_triplet.current.lat = g_takeoff_triplet.current.lat;
    |     o_pos_sp_triplet.current.lon = g_takeoff_triplet.current.lon;
    |     o_pos_sp_triplet.current.yaw = IsFinite(g_takeoff_triplet.current.yaw, o_pos_sp_triplet.current.yaw);
    |     g_takeoff_triplet.current.valid = false;
    | end
    | 
    | % 前一航点
    | o_pos_sp_triplet.previous.valid = false;
    | % 下一航点
    | o_pos_sp_triplet.next.valid = false;
    | 
    | % 置标志位
    | if (isfinite(o_pos_sp_triplet.current.lat) && isfinite(o_pos_sp_triplet.current.lon))
    |     g_can_loiter_at_sp = true;
    | else
    |     g_can_loiter_at_sp = false;
    | end
    | 
    | g_pos_sp_triplet_updated = true;
    | 
    | end
    | 
    | %% 设置takeoff_item
    | function set_takeoff_item(alt)
    | 
    | g_mission_item.nav_cmd = uint16(NAVIGATION_CMD.NAV_CMD_TAKEOFF);
    | g_mission_item.lat = i_global_position.lat;
    | g_mission_item.lon = i_global_position.lon;
    | g_mission_item.yaw = i_local_position.heading;
    | g_mission_item.altitude = alt;
    | g_mission_item.altitude_is_relative = false;
    | g_mission_item.loiter_radius = NAV_LOITER_RAD;
    | g_mission_item.autocontinue = false;
    | g_mission_item.origin = uint8(MISSION_ORIGIN.ONBOARD);
    | 
    | end
  function advance_ef:
    | function advance_ef
    | 
    | switch (ef_state)
    |     
    |     case EFSTATE.EF_STATE_NONE
    |         sprintf("Engine failure. Loitering down. \n")
    |         % mavlink_log_emergency
    |         ef_state = EFSTATE.EF_STATE_LOITERDOWN;
    |         
    |     otherwise
    |         
    | end
    | 
    | end
  function set_ef_item:
    | function set_ef_item
    | 
    | % 由于engine failure，将当前的setpoint设置为上一个setpoint，飞机也不能loiter
    | o_pos_sp_triplet.previous = o_pos_sp_triplet.current;
    | g_can_loiter_at_sp = false;
    | 
    | switch (ef_state)
    |     
    |     case EFSTATE.EF_STATE_LOITERDOWN
    |         % 在飞机的当前位置创建一个mission_item
    |         g_mission_item.lat = i_global_position.lat;
    |         g_mission_item.lon = i_global_position.lon;
    |         g_mission_item.altitude_is_relative = false;
    |         g_mission_item.altitude = single(i_home_position.alt - 1000.0); % setting altitude to a very low value
    |         g_mission_item.yaw = single(nan);
    |         g_mission_item.loiter_radius = NAV_LOITER_RAD;
    |         g_mission_item.nav_cmd = uint16(NAVIGATION_CMD.NAV_CMD_LOITER_UNLIMITED);
    |         g_mission_item.acceptance_radius = navigator.get_acceptance_radius;
    |         g_mission_item.autocontinue = true;
    |         g_mission_item.origin = uint8(MISSION_ORIGIN.ONBOARD);
    |         g_can_loiter_at_sp = true;
    |         
    |     otherwise
    |         
    | end
    | 
    | % reset_mission_item_reached
    | g_waypoint_position_reached = false;
    | waypoint_yaw_reached_ = false;
    | time_wp_reached_ = uint64(0);
    | 
    | % convert mission item to current position setpoint and make it valid
    | mission_item_ = NAV_STATE_ACTION.mission_apply_limitation(g_mission_item);
    | NAV_STATE_ACTION.mission_item_to_position_setpoint(g_mission_item);
    | o_pos_sp_triplet.next.valid = false;
    | 
    | g_pos_sp_triplet_updated = true;
    | 
    | end
  function advance_gpsf:
    | function advance_gpsf
    | 
    | switch (gpsf_state)
    |     
    |     case GPSFSTATE.GPSF_STATE_NONE
    |         gpsf_state = GPSFSTATE.GPSF_STATE_LOITER;
    |         
    |     case GPSFSTATE.GPSF_STATE_LOITER
    |         gpsf_state = GPSFSTATE.GPSF_STATE_TERMINATE;
    |         
    |     case GPSFSTATE.GPSF_STATE_TERMINATE
    |         gpsf_state = GPSFSTATE.GPSF_STATE_END;
    |         
    |     otherwise
    |         
    | end
    |     
    | end
  function set_gpsf_item:
    | function set_gpsf_item
    |  
    | o_pos_sp_triplet.previous.valid = false;
    | o_pos_sp_triplet.current.valid = false;
    | o_pos_sp_triplet.next.valid = false;
    | 
    | switch gpsf_state
    |     
    |     case (GPSFSTATE.GPSF_STATE_TERMINATE)
    |         
    |         o_mission_result.flight_termination = true;
    |         g_mission_result_updated = true;
    |         sprintf("GPS failure: request flight termination. \n")
    |         
    |     otherwise
    |         
    | end
    | 
    | g_pos_sp_triplet_updated = true;
    | 
    | end
  function set_idle_item:
    | function set_idle_item()
    | 
    | g_mission_item.nav_cmd = uint16(0);
    | g_mission_item.lat = i_home_position.lat;
    | g_mission_item.lon = i_home_position.lon;
    | g_mission_item.altitude_is_relative = false;
    | g_mission_item.alt = i_home_position.alt;
    | g_mission_item.yaw = single(nan);
    | g_mission_item.loiter_radius = get_loiter_radius();
    | g_mission_item.acceptance_radius = get_acceptance_radius();
    | g_mission_item.time_inside = single(0.0);
    | g_mission_item.autocontinue = true;
    | g_mission_item.origin = MISSION_ORIGIN_ONBOARD;
    | 
    | end
  function time = get_time_inside(item):
    | function time = get_time_inside(item)
    | 
    | time = single(0);
    | 
    | if ((item.nav_cmd == uint16(MAV_CMD.NAV_WAYPOINT) && ...
    |         i_vehicle_status.vehicle_type == VEHICLE_STATUS.VEHICLE_TYPE_ROTARY_WING) || ....
    |         item.nav_cmd == uint16(MAV_CMD.NAV_LOITER_TIME) || ...
    |         item.nav_cmd == uint16(MAV_CMD.NAV_DELAY))
    |     time = max(item.time_inside, single(0));
    | end
    | 
    | end
  function mission_item_to_position_setpoint:
    | % Convert a mission g_mission_item to a position setpoint
    | function mission_item_to_position_setpoint()
    | 
    | % TO DO: don't change the setpoint for non-position items
    | % if (!item_contains_position(g_mission_item)) {
    | % 		return false;
    | % 	}
    | 
    | o_pos_sp_triplet.current.timestamp = uint64(getSimulationTime()*1e6);
    | o_pos_sp_triplet.current.valid = true;
    | 
    | %% 纬度、经度、高度、航向、航向有效性
    | o_pos_sp_triplet.current.lat = g_mission_item.lat;
    | o_pos_sp_triplet.current.lon = g_mission_item.lon;
    | o_pos_sp_triplet.current.alt = get_absolute_altitude_for_item();
    | o_pos_sp_triplet.current.yaw = g_mission_item.yaw;
    | o_pos_sp_triplet.current.yaw_valid = isfinite(g_mission_item.yaw);
    | 
    | %% 盘旋半径、盘旋方向、提前量
    | o_pos_sp_triplet.current.loiter_radius = selection(abs(g_mission_item.loiter_radius), 0.001, abs(g_mission_item.loiter_radius), NAV_LOITER_RAD);
    | o_pos_sp_triplet.current.loiter_direction = int8(sign(g_mission_item.loiter_radius));
    | if isfinite(g_mission_item.acceptance_radius) && (g_mission_item.acceptance_radius > 0.0)
    |     o_pos_sp_triplet.current.acceptance_radius = g_mission_item.acceptance_radius;
    | else
    |     o_pos_sp_triplet.current.acceptance_radius = NAV_ACC_RAD;
    | end
    | 
    | %% 巡航速度、巡航油门
    | o_pos_sp_triplet.current.cruising_speed = get_cruising_speed();
    | o_pos_sp_triplet.current.cruising_throttle = selection(g_mission_throttle, eps, g_mission_throttle, single(nan));
    | 
    | 
    | %% 设置mission g_mission_item.cmd
    | switch g_mission_item.nav_cmd
    |     
    |     case NAVIGATION_CMD.NAV_CMD_IDLE
    |         o_pos_sp_triplet.current.type = uint8(POSITION_SETPOINT.SETPOINT_TYPE_IDLE);
    |         
    |     case NAVIGATION_CMD.NAV_CMD_TAKEOFF
    |         % if already flying (armed and !landed) treat TAKEOFF like regular POSITION
    |         if ((i_vehicle_status.arming_state == VEHICLE_STATUS.ARMING_STATE_ARMED) && ~land_detected.landed && ~land_detected.maybe_landed)
    |             o_pos_sp_triplet.current.type = uint8(POSITION_SETPOINT.SETPOINT_TYPE_POSITION);
    |         else
    |             o_pos_sp_triplet.current.type = uint8(POSITION_SETPOINT.SETPOINT_TYPE_TAKEOFF);
    |         end
    |         
    |     case NAVIGATION_CMD.NAV_CMD_VTOL_TAKEOFF
    |         o_pos_sp_triplet.current.type = uint8(POSITION_SETPOINT.SETPOINT_TYPE_TAKEOFF);
    |         
    |     case {NAVIGATION_CMD.NAV_CMD_LAND, NAVIGATION_CMD.NAV_CMD_VTOL_LAND} 
    |         o_pos_sp_triplet.current.type = uint8(POSITION_SETPOINT.SETPOINT_TYPE_LAND);
    |         
    |     case NAVIGATION_CMD.NAV_CMD_LOITER_TO_ALT
    |         
    |         o_pos_sp_triplet.current.type = uint8(POSITION_SETPOINT.SETPOINT_TYPE_LOITER);
    |         
    |         % MIS_LTRMIN_ALT：这是飞机需要遵守的最低高度，目的是排除地面效应；设置为-1，如果不应该有最小的loiter高度
    |         if (MIS_LTRMIN_ALT > 0.0)
    |             o_pos_sp_triplet.current.alt = max(i_global_position.alt, i_home_position.alt + MIS_LTRMIN_ALT);
    |         else
    |             o_pos_sp_triplet.current.alt = i_global_position.alt;
    |         end
    | 
    |     case {NAVIGATION_CMD.NAV_CMD_LOITER_TIME_LIMIT, NAVIGATION_CMD.NAV_CMD_LOITER_UNLIMITED}
    |         o_pos_sp_triplet.current.type = uint8(POSITION_SETPOINT.SETPOINT_TYPE_LOITER);
    |         
    |     otherwise
    |         o_pos_sp_triplet.current.type = uint8(POSITION_SETPOINT.SETPOINT_TYPE_POSITION);
    |         
    | end
    | 
    | % o_pos_sp_triplet.current.disable_weather_vane = true;
    | 
    | % %%%%%%%%%%%%%%%%%%%%%%%%%%%%%%%%%%%%%%%%%%%%
    | % o_pos_sp_triplet.current.vx = single(nan);
    | % o_pos_sp_triplet.current.vy = single(nan);
    | % o_pos_sp_triplet.current.vz = single(nan);
    | % o_pos_sp_triplet.current.velocity_valid = false;
    | % o_pos_sp_triplet.current.velocity_frame = uint8(0);
    | % o_pos_sp_triplet.current.alt_valid = true;
    | % 
    | % o_pos_sp_triplet.current.yawspeed = single(nan);
    | % o_pos_sp_triplet.current.yawspeed_valid = false;
    | % o_pos_sp_triplet.current.landing_gear = int8(0);
    | % 
    | 
    | end
  function set_takeoff_item(abs_altitude):
    | function set_takeoff_item(abs_altitude)
    | 
    | g_mission_item.nav_cmd = uint16(MAV_CMD.NAV_TAKEOFF);
    | 
    | % use current position
    | g_mission_item.lat = i_global_position.lat;
    | g_mission_item.lon = i_global_position.lon;
    | g_mission_item.yaw = i_local_position.heading;
    | 
    | g_mission_item.alt = abs_altitude;
    | g_mission_item.altitude_is_relative = false;
    | 
    | g_mission_item.loiter_radius = get_loiter_radius();
    | g_mission_item.autocontinue = false;
    | g_mission_item.origin = MISSION_ORIGIN_ONBOARD;
    | 
    | end
  function alt = get_absolute_altitude_for_item:
    | function alt = get_absolute_altitude_for_item()
    | 
    | 
    | if (g_mission_item.altitude_is_relative)
    |     alt = g_mission_item.alt + i_home_position.alt;
    | else
    |     alt = g_mission_item.alt;
    | end
  function mission_apply_limitation:
    | function mission_apply_limitation()
    | 
    | if (i_land_detected.alt_max > 0.0)
    |     % absolute altitude
    |     if g_mission_item.altitude_is_relative
    |         altitude_abs = g_mission_item.alt + i_home_position.alt;
    |     else
    |         altitude_abs = g_mission_item.alt;
    |     end
    | 
    |     % limit altitude to maximum allowed altitude
    |     if ((i_land_detected.alt_max + i_home_position.alt) < altitude_abs)
    |         if g_mission_item.altitude_is_relative
    |             g_mission_item.alt = i_land_detected.alt_max;
    |         else
    |             g_mission_item.alt = i_land_detected.alt_max+ i_home_position.alt;
    | 
    |         end
    |     end
    | end
  function isreached = is_mission_item_reached:
    | function isreached = is_mission_item_reached()
    | 
    | isreached = false;
    | 
    | % % 处理非导航指令和非定义的航点
    | % switch item.nav_cmd
    | % 
    | %     case uint16(NAVIGATION_CMD.NAV_CMD_DO_SET_SERVO)
    | %         isreached = true;
    | % 
    | %     case {uint16(NAVIGATION_CMD.NAV_CMD_LAND), uint16(NAVIGATION_CMD.NAV_CMD_VTOL_LAND)}
    | %         isreached = land_detected.landed;
    | % 
    | %     case {uint16(NAVIGATION_CMD.NAV_CMD_IDLE), uint16(NAVIGATION_CMD.NAV_CMD_LOITER_UNLIMITED)}
    | %         isreached = false;
    | % 
    | %     case {uint16(NAVIGATION_CMD.NAV_CMD_DO_LAND_START),               uint16(NAVIGATION_CMD.NAV_CMD_DO_TRIGGER_CONTROL), ...
    | %             uint16(NAVIGATION_CMD.NAV_CMD_DO_DIGICAM_CONTROL),          uint16(NAVIGATION_CMD.NAV_CMD_IMAGE_START_CAPTURE), ...
    | %             uint16(NAVIGATION_CMD.NAV_CMD_IMAGE_STOP_CAPTURE),          uint16(NAVIGATION_CMD.NAV_CMD_VIDEO_START_CAPTURE), ...
    | %             uint16(NAVIGATION_CMD.NAV_CMD_VIDEO_STOP_CAPTURE),          uint16(NAVIGATION_CMD.NAV_CMD_DO_CONTROL_VIDEO), ...
    | %             uint16(NAVIGATION_CMD.NAV_CMD_DO_MOUNT_CONFIGURE),          uint16(NAVIGATION_CMD.NAV_CMD_DO_MOUNT_CONTROL), ...
    | %             uint16(NAVIGATION_CMD.NAV_CMD_DO_GIMBAL_MANAGER_PITCHYAW),  uint16(NAVIGATION_CMD.NAV_CMD_DO_GIMBAL_MANAGER_CONFIGURE), ...
    | %             uint16(NAVIGATION_CMD.NAV_CMD_DO_SET_ROI),                  uint16(NAVIGATION_CMD.NAV_CMD_DO_SET_ROI_LOCATION), ...
    | %             uint16(NAVIGATION_CMD.NAV_CMD_DO_SET_ROI_WPNEXT_OFFSET),    uint16(NAVIGATION_CMD.NAV_CMD_DO_SET_ROI_NONE), ...
    | %             uint16(NAVIGATION_CMD.NAV_CMD_DO_SET_CAM_TRIGG_DIST),       uint16(NAVIGATION_CMD.NAV_CMD_OBLIQUE_SURVEY), ...
    | %             uint16(NAVIGATION_CMD.NAV_CMD_DO_SET_CAM_TRIGG_INTERVAL),   uint16(NAVIGATION_CMD.NAV_CMD_SET_CAMERA_MODE), ...
    | %             uint16(NAVIGATION_CMD.NAV_CMD_SET_CAMERA_ZOOM),             uint16(NAVIGATION_CMD.NAV_CMD_SET_CAMERA_FOCUS)}
    | %         isreached = true;
    | % 
    | %     case uint16(NAVIGATION_CMD.NAV_CMD_DO_VTOL_TRANSITION)
    | %         if (item.time_inside == 3)
    | %             isreached = (i_vehicle_status.vehicle_type == VEHICLE_STATUS.VEHICLE_TYPE_ROTARY_WING);
    | %         elseif (item.time_inside == 4)
    | %             isreached = (i_vehicle_status.vehicle_type == VEHICLE_STATUS.VEHICLE_TYPE_FIXED_WING);
    | %         else
    | %             isreached = false;
    | %         end
    | % 
    | %     case {uint16(NAVIGATION_CMD.NAV_CMD_DO_CHANGE_SPEED), uint16(NAVIGATION_CMD.NAV_CMD_DO_SET_HOME)}
    | %         isreached = true;
    | % end
    | % 
    | % %% 如果飞机没有着陆并且还没有到达指定航点
    | % if (~land_detected.landed && ~g_waypoint_position_reached)
    | % 
    | %     % 将mission_item中的高度转换为绝对海平面高度
    | %     mission_item_altitude_amsl = navigator.get_absolute_altitude_for_item(item.altitude_is_relative, item.altitude);
    | %     % 计算到航点的距离
    | %     [dist_xy, dist_z, dist] = get_distance_to_point_global_wgs84(item.lat, item.lon, mission_item_altitude_amsl, ...
    | %         i_global_position.lat, i_global_position.lon, i_global_position.alt);
    | % 
    | %     if ((item.nav_cmd == uint16(NAVIGATION_CMD.NAV_CMD_TAKEOFF)) || (item.nav_cmd == uint16(NAVIGATION_CMD.NAV_CMD_VTOL_TAKEOFF)) && ...
    | %             (i_vehicle_status.vehicle_type == VEHICLE_STATUS.VEHICLE_TYPE_ROTARY_WING))
    | % 
    | %         %% 垂起/多旋翼起飞
    | %         takeoff_alt = selection(item.altitude_is_relative, eps, item.altitude, item.altitude - i_home_position.alt); % 起飞高度换算成对地高度
    | %         altitude_acceptance_radius = get_altitude_acceptance_radius;
    | % 
    | %         if (takeoff_alt > 0.0) && (takeoff_alt < altitude_acceptance_radius)
    | %             altitude_acceptance_radius = takeoff_alt / 2;
    | %         end
    | % 
    | %         % 飞机的高度到达了默认提前量的一半，认为到达了航点
    | %         if (i_global_position.alt > (mission_item_altitude_amsl - altitude_acceptance_radius))
    | %             g_waypoint_position_reached = true;
    | %         end
    | % 
    | %     elseif (i_vehicle_status.vehicle_type == VEHICLE_STATUS.VEHICLE_TYPE_ROVER) && (item.nav_cmd == uint16(NAVIGATION_CMD.NAV_CMD_TAKEOFF))
    | % 
    | %         %% 无人车的先不管
    | % 
    | %     elseif item.nav_cmd == uint16(NAVIGATION_CMD.NAV_CMD_TAKEOFF)
    | % 
    | %         %% 固定翼起飞
    | %         if ((dist >= 0 && dist <= get_acceptance_radius) && (dist_z <= get_altitude_acceptance_radius))
    | %             g_waypoint_position_reached = true;
    | %         end
    | % 
    | %     elseif (i_vehicle_status.vehicle_type == VEHICLE_STATUS.VEHICLE_TYPE_FIXED_WING) && ...
    | %             (item.nav_cmd == uint16(NAVIGATION_CMD.NAV_CMD_LOITER_UNLIMITED) || item.nav_cmd == uint16(NAVIGATION_CMD.NAV_CMD_LOITER_TIME_LIMIT))
    | % 
    | %         %% 固定翼按时间盘旋
    | %         if ((dist >= 0.0) && (dist_xy <= (get_acceptance_radius + abs(item.loiter_radius))) && (dist_z <= get_altitude_acceptance_radius))
    | %             g_waypoint_position_reached = true;
    | %         end
    | % 
    | %     elseif item.nav_cmd == uint16(NAVIGATION_CMD.NAV_CMD_LOITER_TO_ALT)
    | % 
    | %         %% 固定翼盘旋到高度
    | %         % nav_loiter_to_alt只有在loiter中使用任务项高度。
    | %         % 第一次检查海拔基准点是任务定点（这意味着loiter还没有到达）
    | %         if (abs(i_pos_sp_triplet.current.alt - mission_item_altitude_amsl) >= eps)
    | %             [dist_xy1, dist_z1, dist1] = get_distance_to_point_global_wgs84(item.lat, item.lon, i_pos_sp_triplet.current.alt, ...
    | %                 i_global_position.lat, i_global_position.lon, i_global_position.alt);
    | % 
    | %             if ((dist1 >= 0) && (dist_xy1 <= (get_acceptance_radius + abs(item.loiter_radius))) && (dist_z1 <= get_default_altitude_acceptance_radius))
    | %                 o_pos_sp_triplet.current.alt = mission_item_altitude_amsl;
    | %                 o_pos_sp_triplet.current.type = uint8(POSITION_SETPOINT.SETPOINT_TYPE_LOITER);
    | %                 g_pos_sp_triplet_updated = true;
    | %             end
    | % 
    | %         elseif ((dist >= 0.0) && (dist_xy <= (get_acceptance_radius + abs(item.loiter_radius))) && (dist_z <= get_altitude_acceptance_radius))
    | %             g_waypoint_position_reached = true;
    | %         end
    | % 
    | %     elseif (item.nav_cmd == uint16(NAVIGATION_CMD.NAV_CMD_CONDITION_GATE))
    | % 
    | %         %% item中的航点是否在飞机与当前期望航点之间
    | % 
    | %     elseif item.nav_cmd == uint16(NAVIGATION_CMD.NAV_CMD_DELAY)
    | % 
    | %         %% delay
    | %         g_waypoint_position_reached = true;
    | %         waypoint_yaw_reached_ = true;
    | %         time_wp_reached_ = uint64(getSimulationTime()*1e6);
    | % 
    | %     else
    | %         acceptance_radius = get_acceptance_radius;
    | %         if ((i_vehicle_status.vehicle_type == VEHICLE_STATUS.VEHICLE_TYPE_ROTARY_WING) && isfinite(item.acceptance_radius) && (item.acceptance_radius > eps))
    | %             % 新的提前量
    | %             acceptance_radius = item.acceptance_radius;
    | %         end
    | % 
    | %         % for vtol back transition calculate acceptance radius based on time and ground speed
    | %         if ((item.vtol_back_transition) && (i_vehicle_status.vehicle_type == VEHICLE_STATUS.VEHICLE_TYPE_FIXED_WING))
    | %             velocity = sqrt(i_local_position.vx^2 + i_local_position.vy^2);
    | % 
    | %             if ((VT_B_DEC_MSS > eps) && (velocity > eps))
    | %                 acceptance_radius = ((velocity / VT_B_DEC_MSS / 2) * velocity) + VT_B_REV_DEL * velocity;
    | %             end
    | %         end
    | % 
    | %         if ((dist_xy >= 0.0) && (dist_xy <= acceptance_radius) && (dist_z <= get_altitude_acceptance_radius))
    | %             g_waypoint_position_reached = true;
    | %         end
    | %     end
    | % 
    | %     %% 记录航点到达的时间
    | %     if (g_waypoint_position_reached)
    | %         time_wp_reached_ = uint64(getSimulationTime()*1e6);
    | %     end
    | % 
    | %     if (i_vehicle_status.vehicle_type ~= VEHICLE_STATUS.VEHICLE_TYPE_ROTARY_WING)
    | %         % consider yaw reached for fixed-wing
    | %         waypoint_yaw_reached_ = true;
    | %     end
    | % 
    | % end
    | % 
    | % %% 检查所要求的yaw setpoint是否达到（只用于旋翼飞行）
    | % if (g_waypoint_position_reached && ~waypoint_yaw_reached_)
    | %     if i_vehicle_status.vehicle_type == VEHICLE_STATUS.VEHICLE_TYPE_ROTARY_WING && isfinite(get_yaw_acceptance(item.yaw))
    | % 
    | %         % 多旋翼会判断yaw是否到达
    | %         yaw_error = wrap(item.yaw - i_local_position.heading, -pi, pi);
    | % 
    | %         if (abs(yaw_error) < deg2rad(MIS_YAW_ERR) || (MIS_YAW_TMT >= eps && ~item.force_heading))
    | %             waypoint_yaw_reached_ = true;
    | %         end
    | % 
    | %         % 如果航点到达了，但是在规定的时间内没有到达指定的yaw
    | %         if ((~waypoint_yaw_reached_) && (item.force_heading && (MIS_YAW_TMT >= eps)) && ...
    | %                 (uint64(getSimulationTime()*1e6) - time_wp_reached_)/1000 >= MIS_YAW_TMT) % unit s
    | %             % 设置mission失败
    | %             sprintf("unable to reach heading within timeout. \n")
    | %             % set_mission_failure_heading_timeout();
    | %         end
    | %     else
    | %         % 固定翼不需要判断yaw是否到达
    | %         waypoint_yaw_reachead = true;
    | %     end
    | % end
    | % 
    | % %% time是否达到
    | % if (g_waypoint_position_reached && waypoint_yaw_reached_)
    | % 
    | %     % 如果航点到达且航向到达，那么开始判断inside_time是否到达
    | %     time_inside_reached = false;
    | % 
    | %     if (get_time_inside(item) < eps) || ((uint64(getSimulationTime()*1e6) - time_wp_reached_)/1000 >= get_time_inside(item)) % unit s
    | %         % check if the MAV was long enough inside the waypoint orbit
    | %         time_inside_reached = true;
    | %     end
    | % 
    | %     %% 检查是否到达出口（只适用于固定翼飞行）
    | %     exit_heading_reached = false;
    | % 
    | %     if (time_inside_reached)
    | %         % enforce exit heading if in FW, the next wp is valid, the vehicle is currently loitering and either having force_heading set,
    | %         % or if loitering to achieve altitdue at a NAV_CMD_WAYPOINT
    | %         % 如果在FW中执行退出，那么下一个wp是有效的，该飞机目前正在进行loitering，要么有force_heading设置，要么是在NAV_CMD_WAYPOINT上实现altitdue
    | %         enforce_exit_heading = ((i_vehicle_status.vehicle_type ~= VEHICLE_STATUS.VEHICLE_TYPE_ROTARY_WING) && i_pos_sp_triplet.next.valid && ...
    | %             i_pos_sp_triplet.current.type == uint8(POSITION_SETPOINT.SETPOINT_TYPE_LOITER) && ...
    | %             (item.force_heading || item.nav_cmd == uint16(NAVIGATION_CMD.NAV_CMD_WAYPOINT)));
    | % 
    | %         if (enforce_exit_heading)
    | %             % check if heading for exit is reached (only applies for fixed-wing)
    | %             dist_current_next = get_distance_to_next_waypoint(i_pos_sp_triplet.current.lat, i_pos_sp_triplet.current.lon, ...
    | %                 i_pos_sp_triplet.next.lat, i_pos_sp_triplet.next.lon);
    | % 
    | %             if (dist_current_next > 1.2 * NAV_LOITER_RAD)
    | %                 item.yaw = get_bearing_to_next_waypoint(i_global_position.lat, i_global_position.lon, i_pos_sp_triplet.next.lat, i_pos_sp_triplet.next.lon);
    | %                 cog = atan2(i_local_position.vy, i_local_position.vx);
    | %                 yaw_err = wrap(item.yaw - cog, -pi, pi);
    | %             else
    | %                 yaw_err = single(0.0);
    | %             end
    | % 
    | %             if (abs(yaw_err) < deg2rad(MIS_YAW_ERR))
    | %                 exit_heading_reached = true;
    | %             end
    | % 
    | %         else
    | %             exit_heading_reached = true;
    | %         end
    | % 
    | %     end
    | % 
    | %     %% 设置退出飞行路线到下一个地点
    | %     if (exit_heading_reached)
    | %         % set exit flight course to next waypoint
    | %         % 计算当前sp与下一个sp之间的距离
    | %         range = get_distance_to_next_waypoint(i_pos_sp_triplet.current.lat, i_pos_sp_triplet.current.lon, ...
    | %             i_pos_sp_triplet.next.lat, i_pos_sp_triplet.next.lon);
    | % 
    | %         % reset lat/lon of loiter waypoint so vehicle follows a tangent
    | %         % 重置lat/lon的转线点，因此车辆遵循切线
    | %         if (item.loiter_exit_xtrack && i_pos_sp_triplet.next.valid && isfinite(range) && ...
    | %                 (item.nav_cmd == uint16(NAVIGATION_CMD.NAV_CMD_LOITER_TIME_LIMIT) || item.nav_cmd == uint16(NAVIGATION_CMD.NAV_CMD_LOITER_TO_ALT)))
    | % 
    | %             bearing = get_bearing_to_next_waypoint(i_pos_sp_triplet.current.lat, i_pos_sp_triplet.current.lon, i_pos_sp_triplet.next.lat, i_pos_sp_triplet.next.lon);
    | %             ratio = constrain(item.loiter_radius / range, -1, 1);
    | %             inner_angle = pi/2 - asin(ratio);
    | % 
    | %             if (i_pos_sp_triplet.current.loiter_direction > 0.0)
    | %                 bearing = bearing - inner_angle;
    | %             else
    | %                 bearing = bearing + inner_angle;
    | %             end
    | % 
    | %             % Replace current setpoint lat/lon with tangent coordinate
    | %             [o_pos_sp_triplet.current.lat, o_pos_sp_triplet.current.lon] = waypoint_from_heading_and_distance(i_pos_sp_triplet.current.lat, i_pos_sp_triplet.current.lon, ...
    | %                 bearing, abs(i_pos_sp_triplet.current.loiter_radius));
    | %         end
    | % 
    | %         isreached = true;
    | % 
    | %     end
    | % end
    | % 
    | % end
    | %
  function set_loiter_item(min_clearance):
    | function set_loiter_item(min_clearance)
    | 
    | if land_detected.landed
    |     g_mission_item.nav_cmd = uint16(0);
    | else
    |     g_mission_item.nav_cmd = uint16(MAV_CMD.NAV_LOITER_UNLIM);
    |     if (g_can_loiter_at_sp && i_pos_sp_triplet.current.valid)
    |         % 目标点经纬度
    |         g_mission_item.lat = i_pos_sp_triplet.current.lat;
    |         g_mission_item.lon = i_pos_sp_triplet.current.lon;
    |         g_mission_item.altitude = i_pos_sp_triplet.current.alt;
    |     else
    |         % 飞机当前经纬度
    |         g_mission_item.lat = i_global_position.lat;
    |         g_mission_item.lon = i_global_position.lon;
    |         g_mission_item.altitude = i_global_position.alt;
    |         if (min_clearance > 0) && (g_mission_item.altitude < i_home_position.alt + min_clearance)
    |             g_mission_item.altitude = i_home_position.alt + min_clearance;
    |         end
    |     end
    | 
    |     g_mission_item.altitude_is_relative = false;
    |     g_mission_item.yaw = single(nan);
    |     g_mission_item.loiter_radius = get_loiter_radius();
    |     g_mission_item.acceptance_radius = get_acceptance_radius();
    |     g_mission_item.time_inside = single(0);
    |     g_mission_item.autocontinue = false;
    |     g_mission_item.origin = MISSION_ORIGIN_ONBOARD;
    | end
    | 
    | end
  function item = set_idle_item2:
    | function item = set_idle_item2
    | 
    | item.timestamp = uint64(getSimulationTime()*1e6);
    | item.instance_count = uint32(0);
    | item.sequence_current = uint16(0);
    | item.nav_cmd = uint16(NAVIGATION_CMD.IDLE);
    | item.lat = i_home_position.lat;
    | item.lon = i_home_position.lon;
    | item.time_inside = single(0);
    | item.acceptance_radius = get_acceptance_radius;
    | item.loiter_radius = NAV_LOITER_RAD;
    | item.yaw = single(nan);
    | item.altitude = i_home_position.alt;
    | item.frame = uint8(0);
    | item.origin = uint8(MISSION_ORIGIN.ONBOARD);
    | item.loiter_exit_xtrack = false;
    | item.force_heading = false;
    | item.altitude_is_relative = false;
    | item.autocontinue = true;
    | item.vtol_back_transition = false;
    | 
    | end
  function reset_mission_item_reached:
    | function reset_mission_item_reached
    | g_waypoint_position_reached = false;
    | g_waypoint_yaw_reached = false;
    | g_time_wp_reached = single(0);
  function set_land_item(at_current_location):
    | function set_land_item(at_current_location)
    | 
    | % VTOL transition to RW before landing
    | % if (force_vtol())
    | %     vehicle_command_s vcmd = {};
    | %     vcmd.command = NAV_CMD_DO_VTOL_TRANSITION;
    | %     vcmd.param1 = vtol_vehicle_status_s::VEHICLE_VTOL_STATE_MC;
    | %     vcmd.param2 = 0.0f;
    | %     _navigator->publish_vehicle_cmd(&vcmd);
    | % end
    | 
    | % set the land item
    | g_mission_item.nav_cmd = uint16(MAV_CMD.NAV_LAND);
    | 
    | % use current position
    | if (at_current_location)
    |     g_mission_item.lat = nan; %descend at current position
    |     g_mission_item.lon = nan; %descend at current position
    |     g_mission_item.yaw = i_local_position.heading;
    | 
    | else
    |     % use home position
    |     g_mission_item.lat = i_home_position.lat;
    |     g_mission_item.lon = i_home_position.lon;
    |     g_mission_item.yaw = i_home_position.yaw;
    | end
    | 
    | g_mission_item.altitude = 0;
    | g_mission_item.altitude_is_relative = false;
    | g_mission_item.loiter_radius = get_loiter_radius();
    | g_mission_item.acceptance_radius = get_acceptance_radius();
    | g_mission_item.time_inside = 0.0;
    | g_mission_item.autocontinue = true;
    | g_mission_item.origin = MISSION_ORIGIN_ONBOARD;
  function dist = get_distance_2_next_waypoint(lat_now,lon_now,lat_next,lon_next):
    | function dist = get_distance_2_next_waypoint(lat_now,lon_now,lat_next,lon_next)
    |  
    | dist = get_distance_to_next_waypoint(lat_now,lon_now,lat_next,lon_next);
    | 
    | end
  function bearing = get_bearing_2_next_waypoint(lat_now,lon_now,lat_next,lon_next):
    | function bearing = get_bearing_2_next_waypoint(lat_now,lon_now,lat_next,lon_next)
    |  
    | bearing = get_bearing_to_next_waypoint(lat_now,lon_now,lat_next,lon_next);
    | 
    | end
  function speed = get_cruising_speed:
    | function speed = get_cruising_speed
    | 
    | if i_vehicle_status.vehicle_type == VEHICLE_STATUS.VEHICLE_TYPE_ROTARY_WING
    |     if (g_navigation_mode == VEHICLE_STATUS.NAVIGATION_STATE_AUTO_MISSION) && (g_mission_cruising_speed_mc > 0.0)
    |         speed = g_mission_cruising_speed_mc;
    |     else
    |         speed = single(-1);
    |     end
    | else
    |     if (g_navigation_mode == VEHICLE_STATUS.NAVIGATION_STATE_AUTO_MISSION) && (g_mission_cruising_speed_fw > 0.0)
    |         speed = g_mission_cruising_speed_fw;
    |     else
    |         speed = single(-1);
    |     end
    | end
    | 
    | end
  function radius = get_loiter_radius:
    | function radius = get_loiter_radius
    | 
    | radius = NAV_LOITER_RAD;
  function radius = get_altitude_acceptance_radius:
    | function radius = get_altitude_acceptance_radius
    | 
    | radius = get_default_altitude_acceptance_radius();
    | 
    | if i_vehicle_status.vehicle_type == VEHICLE_STATUS.VEHICLE_TYPE_FIXED_WING && i_pos_sp_triplet.next.type == uint8(POSITION_SETPOINT.SETPOINT_TYPE_LAND) && i_pos_sp_triplet.next.valid
    |     % Use separate (tighter) altitude acceptance for clean altitude starting point before landing
    |     radius = NAV_FW_ALTL_RAD;
    | end
    | 
    | end
  function reset_triplets:
    | function reset_triplets
    | 
    | % previous
    | g_pos_sp_triplet.previous.timestamp = uint64(getSimulationTime()*1e6);
    | g_pos_sp_triplet.previous.lat = nan;
    | g_pos_sp_triplet.previous.lon = nan;
    | g_pos_sp_triplet.previous.loiter_radius = get_loiter_radius();
    | g_pos_sp_triplet.previous.acceptance_radius = get_default_acceptance_radius();
    | g_pos_sp_triplet.previous.cruising_speed = get_cruising_speed();
    | g_pos_sp_triplet.previous.cruising_throttle = get_cruising_throttle();
    | g_pos_sp_triplet.previous.valid = false;
    | g_pos_sp_triplet.previous.type = POSITION_SETPOINT.SETPOINT_TYPE_IDLE;
    | g_pos_sp_triplet.previous.disable_weather_vane = false;
    | 
    | % current
    | g_pos_sp_triplet.current.timestamp = uint64(getSimulationTime()*1e6);
    | g_pos_sp_triplet.current.lat = nan;
    | g_pos_sp_triplet.current.lon = nan;
    | g_pos_sp_triplet.current.loiter_radius = get_loiter_radius();
    | g_pos_sp_triplet.current.acceptance_radius = get_default_acceptance_radius();
    | g_pos_sp_triplet.current.cruising_speed = get_cruising_speed();
    | g_pos_sp_triplet.current.cruising_throttle = get_cruising_throttle();
    | g_pos_sp_triplet.current.valid = false;
    | g_pos_sp_triplet.current.type = POSITION_SETPOINT.SETPOINT_TYPE_IDLE;
    | g_pos_sp_triplet.current.disable_weather_vane = false;
    | 
    | % next
    | g_pos_sp_triplet.next.timestamp = uint64(getSimulationTime()*1e6);
    | g_pos_sp_triplet.next.lat = nan;
    | g_pos_sp_triplet.next.lon = nan;
    | g_pos_sp_triplet.next.loiter_radius = get_loiter_radius();
    | g_pos_sp_triplet.next.acceptance_radius = get_default_acceptance_radius();
    | g_pos_sp_triplet.next.cruising_speed = get_cruising_speed();
    | g_pos_sp_triplet.next.cruising_throttle = get_cruising_throttle();
    | g_pos_sp_triplet.next.valid = false;
    | g_pos_sp_triplet.next.type = POSITION_SETPOINT.SETPOINT_TYPE_IDLE;
    | g_pos_sp_triplet.next.disable_weather_vane = false;
  function set_cruising_speed(speed):
    | function set_cruising_speed(speed)
    | 
    | if i_vehicle_status.vehicle_type == VEHICLE_STATUS.VEHICLE_TYPE_ROTARY_WING
    |     g_mission_cruising_speed_mc = speed;
    | else
    |     g_mission_cruising_speed_fw = speed;
    | 
    | end
    | end
  function radius = get_acceptance_radius:
    | function radius = get_acceptance_radius
    | 
    | radius = NAV_ACC_RAD;
    | 
    | % for fixed-wing, return the max of NAV_ACC_RAD and the controller acceptance radius (e.g. L1 distance)
    | if (i_vehicle_status.vehicle_type ~= VEHICLE_STATUS.VEHICLE_TYPE_ROTARY_WING)...
    |     && isfinite(i_pos_ctrl_status.acceptance_radius) && (i_pos_ctrl_status.timestamp ~= 0)
    | 
    |     radius = max(NAV_ACC_RAD, i_pos_ctrl_status.acceptance_radius);
    | end
    | 
    | end
  function radius = get_default_altitude_acceptance_radius:
    | function radius = get_default_altitude_acceptance_radius
    |  
    | if i_vehicle_status.vehicle_type == VEHICLE_STATUS.VEHICLE_TYPE_FIXED_WING
    |     radius = NAV_FW_ALT_RAD;
    | elseif i_vehicle_status.vehicle_type == VEHICLE_STATUS.VEHICLE_TYPE_ROVER
    |     radius = single(Inf);
    | else
    |     alt_acceptance_radius = NAV_MC_ALT_RAD;
    |     if (i_pos_ctrl_status.timestamp > i_pos_sp_triplet.timestamp) && (i_pos_ctrl_status.altitude_acceptance > alt_acceptance_radius)
    |         alt_acceptance_radius = i_pos_ctrl_status.altitude_acceptance;
    |     end
    |     
    |     radius = alt_acceptance_radius;
    | end
    | 
    | end
  function publish_mission_result:
    | function publish_mission_result
    | 
    | o_mission_result.timestamp = hrt_absolute_time();
    | 
    | % lazily publish the mission result only once available
    | % o_mission_result_pub.publish(o_mission_result);
    | 
    | % reset some of the flags
    | o_mission_result.item_do_jump_changed = false;
    | o_mission_result.item_changed_index = 0;
    | o_mission_result.item_do_jump_remaining = 0;
    | 
    | g_mission_result_updated = false;
  function reset_cruising_speed:
    | function reset_cruising_speed()
    | g_mission_cruising_speed_mc = single(-1.0);
    | g_mission_cruising_speed_fw = single(-1.0);
  function radius = get_default_acceptance_radius:
    | function radius = get_default_acceptance_radius
    | radius = NAV_ACC_RAD;
  function yaw = get_yaw_acceptance(mission_item_yaw):
    | function yaw = get_yaw_acceptance(mission_item_yaw)
    | yaw = mission_item_yaw;
    | 
    | % if yaw_acceptance from position controller is NaN overwrite the mission item yaw such that
    | % the waypoint can be reached from any direction
    | if (i_pos_ctrl_status.timestamp > i_pos_sp_triplet.timestamp) && ~isfinite(i_pos_ctrl_status.yaw_acceptance)
    |     yaw = i_pos_ctrl_status.yaw_acceptance;
    | end
    | 
    | end
  function publish_vehicle_command_ack(cmd, result):
    | function publish_vehicle_command_ack(cmd, result)
    |  
    | o_command_ack.timestamp = uint64(getSimulationTime()*1e6);
    | 
    | o_command_ack.command = cmd.command;
    | o_command_ack.target_system = cmd.source_system;
    | o_command_ack.target_component = cmd.source_component;
    | o_command_ack.from_external = false;
    | 
    | o_command_ack.result = uint8(result);
    | o_command_ack.result_param1 = uint8(0);
    | o_command_ack.result_param2 = int32(0);
  function throttle = get_cruising_throttle:
    | function throttle = get_cruising_throttle
    | 
    | if (g_mission_throttle > eps)
    |     throttle = g_mission_throttle;
    | else
    |     throttle = single(nan);
    | end
    | 
    | end
